simulink model "GNC_physical_diagram"  (R2021b)
settings: Solver=VariableStepAuto  StartTime=0.0  StopTime=10.0  RelTol=1e-3
model workspace (MAT data in the model file):
  AV_Status_Signal = Simulink.Bus
  AV_Status_Signal.Alignment = -1
  AV_Status_Signal.PreserveElementDimensions = 0
  AV_Status_Signal.Elements_internal(1) = Simulink.BusElement
  AV_Status_Signal.Elements_internal(1).DimensionsMode = 'Fixed'
  AV_Status_Signal.Elements_internal(1).SamplingMode = 'Sample based'
  AV_Status_Signal.Elements_internal(1).SampleTime = -1
  AV_Status_Signal.Elements_internal(1).Name = 'Detumbling_Trigger'
  AV_Status_Signal.Elements_internal(1).DataType_internal = 'double'
  AV_Status_Signal.Elements_internal(1).Complexity = 'real'
  AV_Status_Signal.Elements_internal(1).Dimensions = 1
  AV_Status_Signal.Elements_internal(2) = Simulink.BusElement
  AV_Status_Signal.Elements_internal(2).DimensionsMode = 'Fixed'
  AV_Status_Signal.Elements_internal(2).SamplingMode = 'Sample based'
  AV_Status_Signal.Elements_internal(2).SampleTime = -1
  AV_Status_Signal.Elements_internal(2).Name = 'Testing_Trigger'
  AV_Status_Signal.Elements_internal(2).DataType_internal = 'double'
  AV_Status_Signal.Elements_internal(2).Complexity = 'real'
  AV_Status_Signal.Elements_internal(2).Dimensions = 1
  AV_Status_Signal.Elements_internal(3) = Simulink.BusElement
  AV_Status_Signal.Elements_internal(3).DimensionsMode = 'Fixed'
  AV_Status_Signal.Elements_internal(3).SamplingMode = 'Sample based'
  AV_Status_Signal.Elements_internal(3).SampleTime = -1
  AV_Status_Signal.Elements_internal(3).Name = 'Rotation_Trigger'
  AV_Status_Signal.Elements_internal(3).DataType_internal = 'double'
  AV_Status_Signal.Elements_internal(3).Complexity = 'real'
  AV_Status_Signal.Elements_internal(3).Dimensions = 1
  AV_Status_Signal.Elements_internal(4) = Simulink.BusElement
  AV_Status_Signal.Elements_internal(4).DimensionsMode = 'Fixed'
  AV_Status_Signal.Elements_internal(4).SamplingMode = 'Sample based'
  AV_Status_Signal.Elements_internal(4).SampleTime = -1
  AV_Status_Signal.Elements_internal(4).Name = 'Recreation_Trigger'
  AV_Status_Signal.Elements_internal(4).DataType_internal = 'double'
  AV_Status_Signal.Elements_internal(4).Complexity = 'real'
  AV_Status_Signal.Elements_internal(4).Dimensions = 1
  AV_Status_Signal.Elements_internal(5) = Simulink.BusElement
  AV_Status_Signal.Elements_internal(5).DimensionsMode = 'Fixed'
  AV_Status_Signal.Elements_internal(5).SamplingMode = 'Sample based'
  AV_Status_Signal.Elements_internal(5).SampleTime = -1
  AV_Status_Signal.Elements_internal(5).Name = 'Maintain_Trigger'
  AV_Status_Signal.Elements_internal(5).DataType_internal = 'double'
  AV_Status_Signal.Elements_internal(5).Complexity = 'real'
  AV_Status_Signal.Elements_internal(5).Dimensions = 1
  AV_Status_Signal.Elements_internal(6) = Simulink.BusElement
  AV_Status_Signal.Elements_internal(6).DimensionsMode = 'Fixed'
  AV_Status_Signal.Elements_internal(6).SamplingMode = 'Sample based'
  AV_Status_Signal.Elements_internal(6).SampleTime = -1
  AV_Status_Signal.Elements_internal(6).Name = 'End_of_Life_Trigger'
  AV_Status_Signal.Elements_internal(6).DataType_internal = 'double'
  AV_Status_Signal.Elements_internal(6).Complexity = 'real'
  AV_Status_Signal.Elements_internal(6).Dimensions = 1
  AV_Status_Signal.DataScope = 'Auto'
  Actuator_Signal = Simulink.Bus
  Actuator_Signal.Alignment = -1
  Actuator_Signal.PreserveElementDimensions = 0
  Actuator_Signal.Elements_internal(1) = Simulink.BusElement
  Actuator_Signal.Elements_internal(1).DimensionsMode = 'Fixed'
  Actuator_Signal.Elements_internal(1).SamplingMode = 'Sample based'
  Actuator_Signal.Elements_internal(1).SampleTime = -1
  Actuator_Signal.Elements_internal(1).Name = 'Reaction_Wheel_Signal'
  Actuator_Signal.Elements_internal(1).DataType_internal = 'double'
  Actuator_Signal.Elements_internal(1).Complexity = 'real'
  Actuator_Signal.Elements_internal(1).Dimensions = 1
  Actuator_Signal.Elements_internal(2) = Simulink.BusElement
  Actuator_Signal.Elements_internal(2).DimensionsMode = 'Fixed'
  Actuator_Signal.Elements_internal(2).SamplingMode = 'Sample based'
  Actuator_Signal.Elements_internal(2).SampleTime = -1
  Actuator_Signal.Elements_internal(2).Name = 'Magnetorquer_Signal'
  Actuator_Signal.Elements_internal(2).DataType_internal = 'double'
  Actuator_Signal.Elements_internal(2).Complexity = 'real'
  Actuator_Signal.Elements_internal(2).Dimensions = 1
  Actuator_Signal.DataScope = 'Auto'
  Data_Stream = Simulink.Bus
  Data_Stream.Alignment = -1
  Data_Stream.PreserveElementDimensions = 0
  Data_Stream.Elements_internal(1) = Simulink.BusElement
  Data_Stream.Elements_internal(1).DimensionsMode = 'Fixed'
  Data_Stream.Elements_internal(1).SamplingMode = 'Sample based'
  Data_Stream.Elements_internal(1).SampleTime = -1
  Data_Stream.Elements_internal(1).Name = 'State_Estimation_Data'
  Data_Stream.Elements_internal(1).DataType_internal = 'double'
  Data_Stream.Elements_internal(1).Complexity = 'real'
  Data_Stream.Elements_internal(1).Dimensions = 1
  Data_Stream.Elements_internal(2) = Simulink.BusElement
  Data_Stream.Elements_internal(2).DimensionsMode = 'Fixed'
  Data_Stream.Elements_internal(2).SamplingMode = 'Sample based'
  Data_Stream.Elements_internal(2).SampleTime = -1
  Data_Stream.Elements_internal(2).Name = 'Output_Mission_Phases'
  Data_Stream.Elements_internal(2).DataType_internal = 'double'
  Data_Stream.Elements_internal(2).Complexity = 'real'
  Data_Stream.Elements_internal(2).Dimensions = 1
  Data_Stream.Elements_internal(3) = Simulink.BusElement
  Data_Stream.Elements_internal(3).DimensionsMode = 'Fixed'
  Data_Stream.Elements_internal(3).SamplingMode = 'Sample based'
  Data_Stream.Elements_internal(3).SampleTime = -1
  Data_Stream.Elements_internal(3).Name = 'Encoder_Data'
  Data_Stream.Elements_internal(3).DataType_internal = 'double'
  Data_Stream.Elements_internal(3).Complexity = 'real'
  Data_Stream.Elements_internal(3).Dimensions = 1
  Data_Stream.Elements_internal(4) = Simulink.BusElement
  Data_Stream.Elements_internal(4).DimensionsMode = 'Fixed'
  Data_Stream.Elements_internal(4).SamplingMode = 'Sample based'
  Data_Stream.Elements_internal(4).SampleTime = -1
  Data_Stream.Elements_internal(4).Name = 'Sensor_Fusion'
  Data_Stream.Elements_internal(4).DataType_internal = 'double'
  Data_Stream.Elements_internal(4).Complexity = 'real'
  Data_Stream.Elements_internal(4).Dimensions = 1
  Data_Stream.DataScope = 'Auto'
  Magnetororquer_Signal = Simulink.Bus
  Magnetororquer_Signal.Alignment = -1
  Magnetororquer_Signal.PreserveElementDimensions = 0
  Magnetororquer_Signal.Elements_internal(1) = Simulink.BusElement
  Magnetororquer_Signal.Elements_internal(1).DimensionsMode = 'Fixed'
  Magnetororquer_Signal.Elements_internal(1).SamplingMode = 'Sample based'
  Magnetororquer_Signal.Elements_internal(1).SampleTime = -1
  Magnetororquer_Signal.Elements_internal(1).Name = 'Magnetororquer_1_Signal'
  Magnetororquer_Signal.Elements_internal(1).DataType_internal = 'double'
  Magnetororquer_Signal.Elements_internal(1).Complexity = 'real'
  Magnetororquer_Signal.Elements_internal(1).Dimensions = 1
  Magnetororquer_Signal.Elements_internal(2) = Simulink.BusElement
  Magnetororquer_Signal.Elements_internal(2).DimensionsMode = 'Fixed'
  Magnetororquer_Signal.Elements_internal(2).SamplingMode = 'Sample based'
  Magnetororquer_Signal.Elements_internal(2).SampleTime = -1
  Magnetororquer_Signal.Elements_internal(2).Name = 'Magnetororquer_2_Signal'
  Magnetororquer_Signal.Elements_internal(2).DataType_internal = 'double'
  Magnetororquer_Signal.Elements_internal(2).Complexity = 'real'
  Magnetororquer_Signal.Elements_internal(2).Dimensions = 1
  Magnetororquer_Signal.Elements_internal(3) = Simulink.BusElement
  Magnetororquer_Signal.Elements_internal(3).DimensionsMode = 'Fixed'
  Magnetororquer_Signal.Elements_internal(3).SamplingMode = 'Sample based'
  Magnetororquer_Signal.Elements_internal(3).SampleTime = -1
  Magnetororquer_Signal.Elements_internal(3).Name = 'Magnetororquer_3_Signal'
  Magnetororquer_Signal.Elements_internal(3).DataType_internal = 'double'
  Magnetororquer_Signal.Elements_internal(3).Complexity = 'real'
  Magnetororquer_Signal.Elements_internal(3).Dimensions = 1
  Magnetororquer_Signal.Elements_internal(4) = Simulink.BusElement
  Magnetororquer_Signal.Elements_internal(4).DimensionsMode = 'Fixed'
  Magnetororquer_Signal.Elements_internal(4).SamplingMode = 'Sample based'
  Magnetororquer_Signal.Elements_internal(4).SampleTime = -1
  Magnetororquer_Signal.Elements_internal(4).Name = 'Magnetororquer_4_Signal'
  Magnetororquer_Signal.Elements_internal(4).DataType_internal = 'double'
  Magnetororquer_Signal.Elements_internal(4).Complexity = 'real'
  Magnetororquer_Signal.Elements_internal(4).Dimensions = 1
  Magnetororquer_Signal.DataScope = 'Auto'
  Mode_Trigger = Simulink.Bus
  Mode_Trigger.Alignment = -1
  Mode_Trigger.PreserveElementDimensions = 0
  Mode_Trigger.Elements_internal(1) = Simulink.BusElement
  Mode_Trigger.Elements_internal(1).DimensionsMode = 'Fixed'
  Mode_Trigger.Elements_internal(1).SamplingMode = 'Sample based'
  Mode_Trigger.Elements_internal(1).SampleTime = -1
  Mode_Trigger.Elements_internal(1).Name = 'Low_Gravity_Mode_Trigger'
  Mode_Trigger.Elements_internal(1).DataType_internal = 'double'
  Mode_Trigger.Elements_internal(1).Complexity = 'real'
  Mode_Trigger.Elements_internal(1).Dimensions = 1
  Mode_Trigger.Elements_internal(2) = Simulink.BusElement
  Mode_Trigger.Elements_internal(2).DimensionsMode = 'Fixed'
  Mode_Trigger.Elements_internal(2).SamplingMode = 'Sample based'
  Mode_Trigger.Elements_internal(2).SampleTime = -1
  Mode_Trigger.Elements_internal(2).Name = 'High_Gravity_Trigger'
  Mode_Trigger.Elements_internal(2).DataType_internal = 'double'
  Mode_Trigger.Elements_internal(2).Complexity = 'real'
  Mode_Trigger.Elements_internal(2).Dimensions = 1
  Mode_Trigger.Elements_internal(3) = Simulink.BusElement
  Mode_Trigger.Elements_internal(3).DimensionsMode = 'Fixed'
  Mode_Trigger.Elements_internal(3).SamplingMode = 'Sample based'
  Mode_Trigger.Elements_internal(3).SampleTime = -1
  Mode_Trigger.Elements_internal(3).Name = 'Desaturization_Trigger'
  Mode_Trigger.Elements_internal(3).DataType_internal = 'double'
  Mode_Trigger.Elements_internal(3).Complexity = 'real'
  Mode_Trigger.Elements_internal(3).Dimensions = 1
  Mode_Trigger.Elements_internal(4) = Simulink.BusElement
  Mode_Trigger.Elements_internal(4).DimensionsMode = 'Fixed'
  Mode_Trigger.Elements_internal(4).SamplingMode = 'Sample based'
  Mode_Trigger.Elements_internal(4).SampleTime = -1
  Mode_Trigger.Elements_internal(4).Name = 'Safe_Mode_Trigger'
  Mode_Trigger.Elements_internal(4).DataType_internal = 'double'
  Mode_Trigger.Elements_internal(4).Complexity = 'real'
  Mode_Trigger.Elements_internal(4).Dimensions = 1
  Mode_Trigger.Elements_internal(5) = Simulink.BusElement
  Mode_Trigger.Elements_internal(5).DimensionsMode = 'Fixed'
  Mode_Trigger.Elements_internal(5).SamplingMode = 'Sample based'
  Mode_Trigger.Elements_internal(5).SampleTime = -1
  Mode_Trigger.Elements_internal(5).Name = 'Collision_Avoidance_Mode'
  Mode_Trigger.Elements_internal(5).DataType_internal = 'double'
  Mode_Trigger.Elements_internal(5).Complexity = 'real'
  Mode_Trigger.Elements_internal(5).Dimensions = 1
  Mode_Trigger.Elements_internal(6) = Simulink.BusElement
  Mode_Trigger.Elements_internal(6).DimensionsMode = 'Fixed'
  Mode_Trigger.Elements_internal(6).SamplingMode = 'Sample based'
  Mode_Trigger.Elements_internal(6).SampleTime = -1
  Mode_Trigger.Elements_internal(6).Name = 'Idle_Mode_Trigger'
  Mode_Trigger.Elements_internal(6).DataType_internal = 'double'
  Mode_Trigger.Elements_internal(6).Complexity = 'real'
  Mode_Trigger.Elements_internal(6).Dimensions = 1
  Mode_Trigger.DataScope = 'Auto'
  Reaction_Wheel_Signal = Simulink.Bus
  Reaction_Wheel_Signal.Alignment = -1
  Reaction_Wheel_Signal.PreserveElementDimensions = 0
  Reaction_Wheel_Signal.Elements_internal(1) = Simulink.BusElement
  Reaction_Wheel_Signal.Elements_internal(1).DimensionsMode = 'Fixed'
  Reaction_Wheel_Signal.Elements_internal(1).SamplingMode = 'Sample based'
  Reaction_Wheel_Signal.Elements_internal(1).SampleTime = -1
  Reaction_Wheel_Signal.Elements_internal(1).Name = 'Reaction_Wheel_1_Signal'
  Reaction_Wheel_Signal.Elements_internal(1).DataType_internal = 'double'
  Reaction_Wheel_Signal.Elements_internal(1).Complexity = 'real'
  Reaction_Wheel_Signal.Elements_internal(1).Dimensions = 1
  Reaction_Wheel_Signal.Elements_internal(2) = Simulink.BusElement
  Reaction_Wheel_Signal.Elements_internal(2).DimensionsMode = 'Fixed'
  Reaction_Wheel_Signal.Elements_internal(2).SamplingMode = 'Sample based'
  Reaction_Wheel_Signal.Elements_internal(2).SampleTime = -1
  Reaction_Wheel_Signal.Elements_internal(2).Name = 'Reaction_Wheel_2_Signal'
  Reaction_Wheel_Signal.Elements_internal(2).DataType_internal = 'double'
  Reaction_Wheel_Signal.Elements_internal(2).Complexity = 'real'
  Reaction_Wheel_Signal.Elements_internal(2).Dimensions = 1
  Reaction_Wheel_Signal.Elements_internal(3) = Simulink.BusElement
  Reaction_Wheel_Signal.Elements_internal(3).DimensionsMode = 'Fixed'
  Reaction_Wheel_Signal.Elements_internal(3).SamplingMode = 'Sample based'
  Reaction_Wheel_Signal.Elements_internal(3).SampleTime = -1
  Reaction_Wheel_Signal.Elements_internal(3).Name = 'Reaction_Wheel_3_Signal'
  Reaction_Wheel_Signal.Elements_internal(3).DataType_internal = 'double'
  Reaction_Wheel_Signal.Elements_internal(3).Complexity = 'real'
  Reaction_Wheel_Signal.Elements_internal(3).Dimensions = 1
  Reaction_Wheel_Signal.Elements_internal(4) = Simulink.BusElement
  Reaction_Wheel_Signal.Elements_internal(4).DimensionsMode = 'Fixed'
  Reaction_Wheel_Signal.Elements_internal(4).SamplingMode = 'Sample based'
  Reaction_Wheel_Signal.Elements_internal(4).SampleTime = -1
  Reaction_Wheel_Signal.Elements_internal(4).Name = 'Reaction_Wheel_4_Signal'
  Reaction_Wheel_Signal.Elements_internal(4).DataType_internal = 'double'
  Reaction_Wheel_Signal.Elements_internal(4).Complexity = 'real'
  Reaction_Wheel_Signal.Elements_internal(4).Dimensions = 1
  Reaction_Wheel_Signal.DataScope = 'Auto'
  Resources_Budget = Simulink.Bus
  Resources_Budget.Alignment = -1
  Resources_Budget.PreserveElementDimensions = 0
  Resources_Budget.Elements_internal(1) = Simulink.BusElement
  Resources_Budget.Elements_internal(1).DimensionsMode = 'Fixed'
  Resources_Budget.Elements_internal(1).SamplingMode = 'Sample based'
  Resources_Budget.Elements_internal(1).SampleTime = -1
  Resources_Budget.Elements_internal(1).Name = 'Processing_Power'
  Resources_Budget.Elements_internal(1).DataType_internal = 'double'
  Resources_Budget.Elements_internal(1).Complexity = 'real'
  Resources_Budget.Elements_internal(1).Dimensions = 1
  Resources_Budget.Elements_internal(2) = Simulink.BusElement
  Resources_Budget.Elements_internal(2).DimensionsMode = 'Fixed'
  Resources_Budget.Elements_internal(2).SamplingMode = 'Sample based'
  Resources_Budget.Elements_internal(2).SampleTime = -1
  Resources_Budget.Elements_internal(2).Name = 'Memory_Allocation'
  Resources_Budget.Elements_internal(2).DataType_internal = 'double'
  Resources_Budget.Elements_internal(2).Complexity = 'real'
  Resources_Budget.Elements_internal(2).Dimensions = 1
  Resources_Budget.Elements_internal(3) = Simulink.BusElement
  Resources_Budget.Elements_internal(3).DimensionsMode = 'Fixed'
  Resources_Budget.Elements_internal(3).SamplingMode = 'Sample based'
  Resources_Budget.Elements_internal(3).SampleTime = -1
  Resources_Budget.Elements_internal(3).Name = 'Power'
  Resources_Budget.Elements_internal(3).DataType_internal = 'double'
  Resources_Budget.Elements_internal(3).Complexity = 'real'
  Resources_Budget.Elements_internal(3).Dimensions = 1
  Resources_Budget.DataScope = 'Auto'
  Sensor_Health = Simulink.Bus
  Sensor_Health.Alignment = -1
  Sensor_Health.PreserveElementDimensions = 0
  Sensor_Health.Elements_internal(1) = Simulink.BusElement
  Sensor_Health.Elements_internal(1).DimensionsMode = 'Fixed'
  Sensor_Health.Elements_internal(1).SamplingMode = 'Sample based'
  Sensor_Health.Elements_internal(1).SampleTime = -1
  Sensor_Health.Elements_internal(1).Name = 'Sun_Sensor_Health'
  Sensor_Health.Elements_internal(1).DataType_internal = 'double'
  Sensor_Health.Elements_internal(1).Complexity = 'real'
  Sensor_Health.Elements_internal(1).Dimensions = 1
  Sensor_Health.Elements_internal(2) = Simulink.BusElement
  Sensor_Health.Elements_internal(2).DimensionsMode = 'Fixed'
  Sensor_Health.Elements_internal(2).SamplingMode = 'Sample based'
  Sensor_Health.Elements_internal(2).SampleTime = -1
  Sensor_Health.Elements_internal(2).Name = 'IMU_Health'
  Sensor_Health.Elements_internal(2).DataType_internal = 'double'
  Sensor_Health.Elements_internal(2).Complexity = 'real'
  Sensor_Health.Elements_internal(2).Dimensions = 1
  Sensor_Health.Elements_internal(3) = Simulink.BusElement
  Sensor_Health.Elements_internal(3).DimensionsMode = 'Fixed'
  Sensor_Health.Elements_internal(3).SamplingMode = 'Sample based'
  Sensor_Health.Elements_internal(3).SampleTime = -1
  Sensor_Health.Elements_internal(3).Name = 'Magnetometer_Health'
  Sensor_Health.Elements_internal(3).DataType_internal = 'double'
  Sensor_Health.Elements_internal(3).Complexity = 'real'
  Sensor_Health.Elements_internal(3).Dimensions = 1
  Sensor_Health.Elements_internal(4) = Simulink.BusElement
  Sensor_Health.Elements_internal(4).DimensionsMode = 'Fixed'
  Sensor_Health.Elements_internal(4).SamplingMode = 'Sample based'
  Sensor_Health.Elements_internal(4).SampleTime = -1
  Sensor_Health.Elements_internal(4).Name = 'GPS_Health'
  Sensor_Health.Elements_internal(4).DataType_internal = 'double'
  Sensor_Health.Elements_internal(4).Complexity = 'real'
  Sensor_Health.Elements_internal(4).Dimensions = 1
  Sensor_Health.DataScope = 'Auto'
  Sensor_Signal = Simulink.Bus
  Sensor_Signal.Alignment = -1
  Sensor_Signal.PreserveElementDimensions = 0
  Sensor_Signal.Elements_internal(1) = Simulink.BusElement
  Sensor_Signal.Elements_internal(1).DimensionsMode = 'Fixed'
  Sensor_Signal.Elements_internal(1).SamplingMode = 'Sample based'
  Sensor_Signal.Elements_internal(1).SampleTime = -1
  Sensor_Signal.Elements_internal(1).Name = 'Sun_Sensor_Measurment'
  Sensor_Signal.Elements_internal(1).DataType_internal = 'double'
  Sensor_Signal.Elements_internal(1).Complexity = 'real'
  Sensor_Signal.Elements_internal(1).Dimensions = 1
  Sensor_Signal.Elements_internal(2) = Simulink.BusElement
  Sensor_Signal.Elements_internal(2).DimensionsMode = 'Fixed'
  Sensor_Signal.Elements_internal(2).SamplingMode = 'Sample based'
  Sensor_Signal.Elements_internal(2).SampleTime = -1
  Sensor_Signal.Elements_internal(2).Name = 'IMU_Measurement'
  Sensor_Signal.Elements_internal(2).DataType_internal = 'double'
  Sensor_Signal.Elements_internal(2).Complexity = 'real'
  Sensor_Signal.Elements_internal(2).Dimensions = 1
  Sensor_Signal.Elements_internal(3) = Simulink.BusElement
  Sensor_Signal.Elements_internal(3).DimensionsMode = 'Fixed'
  Sensor_Signal.Elements_internal(3).SamplingMode = 'Sample based'
  Sensor_Signal.Elements_internal(3).SampleTime = -1
  Sensor_Signal.Elements_internal(3).Name = 'Magnetometer_Measurement'
  Sensor_Signal.Elements_internal(3).DataType_internal = 'double'
  Sensor_Signal.Elements_internal(3).Complexity = 'real'
  Sensor_Signal.Elements_internal(3).Dimensions = 1
  Sensor_Signal.Elements_internal(4) = Simulink.BusElement
  Sensor_Signal.Elements_internal(4).DimensionsMode = 'Fixed'
  Sensor_Signal.Elements_internal(4).SamplingMode = 'Sample based'
  Sensor_Signal.Elements_internal(4).SampleTime = -1
  Sensor_Signal.Elements_internal(4).Name = 'GPS_Measurement'
  Sensor_Signal.Elements_internal(4).DataType_internal = 'double'
  Sensor_Signal.Elements_internal(4).Complexity = 'real'
  Sensor_Signal.Elements_internal(4).Dimensions = 1
  Sensor_Signal.DataScope = 'Auto'
(part 1 of 2)
settings Model: Creator=jonas  LastModifiedBy=leoba

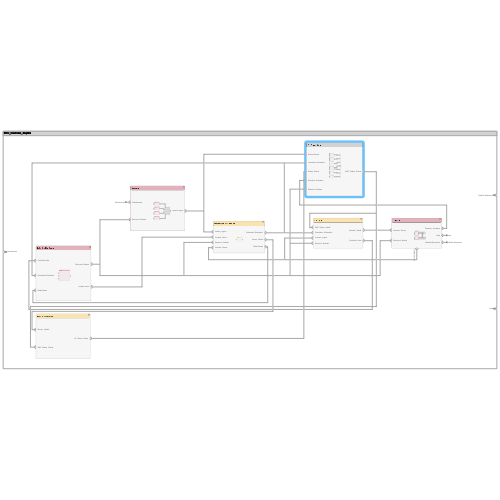
[thumbnail: Simulink's stored preview of the top-level diagram]
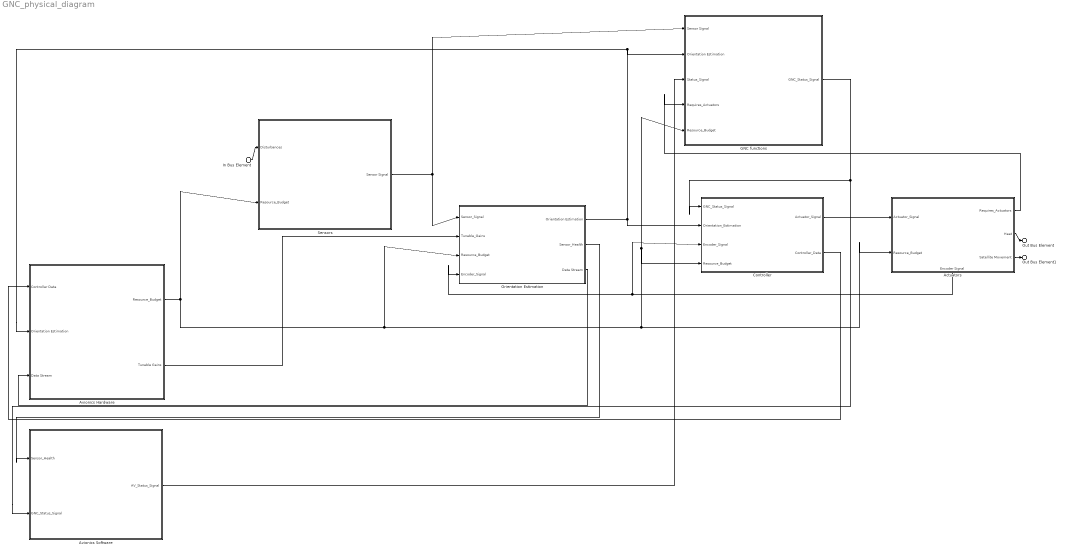
== system GNC_physical_diagram ==
  In Bus Element : Inport  PortName=Disturbances
  Actuators : Subsystem
      settings: PortSchema="{\"entries\":[{\"content\":{\"headerSize\":26,\"margin\":15,\"minimumSpacing\":25,\"sides\":[{\"content\":{\"connectorIds\":[\"In1\",\"In2\"]},\"type\":\"ConnectorPlacement.EquallySpacedRectSide\",\"uuid\":\"4d219d8c-999e-4fa6-ade9-cc6ac14ded32\"},{\"content\":{\"connectorIds\":[\"Out1\",\"Out2\",\"Out3\"],\"side\":\"RIGHT\"},\"type\":\"ConnectorPlacement.EquallySpacedRectSide\",\"uuid\":\"291554bf-cd30-4ae6-93e5-4052e0d4037d\"},{\"content\":{\"connectorIds\":[],\"side\":\"TOP\"},\"type\":\"ConnectorPlacement.EquallySpacedRectSide\",\"uuid\":\"a407b5ba-b8ce-49a8-af7c-64b4689399b6\"},{\"content\":{\"connectorIds\":[\"Out4\"],\"side\":\"BOTTOM\"},\"type\":\"ConnectorPlacement.EquallySpacedRectSide\",\"uuid\":\"28acc806-9e86-4bc6-af71-2b4411156648\"}]},\"type\":\"ConnectorPlacement.EquallySpacedConnector\",\"uuid\":\"1a65b071-c199-4364-8343-b80f4df9252b\"}],\"packageUris\":[\"http://schema.mathworks.com/mf0/Connector/R2020b\"],\"version\":\"1.0\"}"
  Avionics Hardware : Subsystem
      settings: PortSchema="{\"entries\":[{\"content\":{\"headerSize\":26,\"margin\":15,\"minimumSpacing\":25,\"sides\":[{\"content\":{\"connectorIds\":[\"In1\",\"In3\",\"In2\"]},\"type\":\"ConnectorPlacement.EquallySpacedRectSide\",\"uuid\":\"4d219d8c-999e-4fa6-ade9-cc6ac14ded32\"},{\"content\":{\"connectorIds\":[\"Out1\",\"Out2\"],\"side\":\"RIGHT\"},\"type\":\"ConnectorPlacement.EquallySpacedRectSide\",\"uuid\":\"291554bf-cd30-4ae6-93e5-4052e0d4037d\"},{\"content\":{\"connectorIds\":[],\"side\":\"TOP\"},\"type\":\"ConnectorPlacement.EquallySpacedRectSide\",\"uuid\":\"a407b5ba-b8ce-49a8-af7c-64b4689399b6\"},{\"content\":{\"connectorIds\":[],\"side\":\"BOTTOM\"},\"type\":\"ConnectorPlacement.EquallySpacedRectSide\",\"uuid\":\"eed5de48-d554-4a4a-aaed-8ac1beb8b61e\"}]},\"type\":\"ConnectorPlacement.EquallySpacedConnector\",\"uuid\":\"1a65b071-c199-4364-8343-b80f4df9252b\"}],\"packageUris\":[\"http://schema.mathworks.com/mf0/Connector/R2020b\"],\"version\":\"1.0\"}"
  Avionics Software : Subsystem
      settings: PortSchema="{\"entries\":[{\"content\":{\"headerSize\":26,\"margin\":15,\"minimumSpacing\":25,\"sides\":[{\"content\":{\"connectorIds\":[\"In1\",\"In2\"]},\"type\":\"ConnectorPlacement.EquallySpacedRectSide\",\"uuid\":\"9c9f921c-2c3b-482c-ae0a-30fa5cf19172\"},{\"content\":{\"connectorIds\":[\"Out1\"],\"side\":\"RIGHT\"},\"type\":\"ConnectorPlacement.EquallySpacedRectSide\",\"uuid\":\"566c4868-5865-4e1f-981e-d74a35c979c9\"},{\"content\":{\"connectorIds\":[],\"side\":\"TOP\"},\"type\":\"ConnectorPlacement.EquallySpacedRectSide\",\"uuid\":\"2cd88ae2-a2e5-4e25-b817-9d229c73c4c9\"}]},\"type\":\"ConnectorPlacement.EquallySpacedConnector\",\"uuid\":\"48eadbd9-1de4-4fec-af56-45dc4412e923\"}],\"packageUris\":[\"http://schema.mathworks.com/mf0/Connector/R2020b\"],\"version\":\"1.0\"}"
  Controller : Subsystem
      settings: PortSchema="{\"entries\":[{\"content\":{\"headerSize\":26,\"margin\":15,\"minimumSpacing\":25,\"sides\":[{\"content\":{\"connectorIds\":[\"In1\",\"In2\",\"In3\",\"In4\"]},\"type\":\"ConnectorPlacement.EquallySpacedRectSide\",\"uuid\":\"4d219d8c-999e-4fa6-ade9-cc6ac14ded32\"},{\"content\":{\"connectorIds\":[\"Out1\",\"Out2\"],\"side\":\"RIGHT\"},\"type\":\"ConnectorPlacement.EquallySpacedRectSide\",\"uuid\":\"291554bf-cd30-4ae6-93e5-4052e0d4037d\"},{\"content\":{\"connectorIds\":[],\"side\":\"TOP\"},\"type\":\"ConnectorPlacement.EquallySpacedRectSide\",\"uuid\":\"a407b5ba-b8ce-49a8-af7c-64b4689399b6\"}]},\"type\":\"ConnectorPlacement.EquallySpacedConnector\",\"uuid\":\"1a65b071-c199-4364-8343-b80f4df9252b\"}],\"packageUris\":[\"http://schema.mathworks.com/mf0/Connector/R2020b\"],\"version\":\"1.0\"}"
  GNC functions : Subsystem
      settings: PortSchema="{\"entries\":[{\"content\":{\"headerSize\":26,\"margin\":15,\"minimumSpacing\":25,\"sides\":[{\"content\":{\"connectorIds\":[\"In1\",\"In2\",\"In3\",\"In4\",\"In5\"]},\"type\":\"ConnectorPlacement.EquallySpacedRectSide\",\"uuid\":\"9c9f921c-2c3b-482c-ae0a-30fa5cf19172\"},{\"content\":{\"connectorIds\":[\"Out1\"],\"side\":\"RIGHT\"},\"type\":\"ConnectorPlacement.EquallySpacedRectSide\",\"uuid\":\"566c4868-5865-4e1f-981e-d74a35c979c9\"},{\"content\":{\"connectorIds\":[],\"side\":\"TOP\"},\"type\":\"ConnectorPlacement.EquallySpacedRectSide\",\"uuid\":\"2cd88ae2-a2e5-4e25-b817-9d229c73c4c9\"}]},\"type\":\"ConnectorPlacement.EquallySpacedConnector\",\"uuid\":\"48eadbd9-1de4-4fec-af56-45dc4412e923\"}],\"packageUris\":[\"http://schema.mathworks.com/mf0/Connector/R2020b\"],\"version\":\"1.0\"}"
  Orientation Estimation : Subsystem
      settings: PortSchema="{\"entries\":[{\"content\":{\"headerSize\":26,\"margin\":15,\"minimumSpacing\":25,\"sides\":[{\"content\":{\"connectorIds\":[\"In1\",\"In2\",\"In3\",\"In4\"]},\"type\":\"ConnectorPlacement.EquallySpacedRectSide\",\"uuid\":\"4d219d8c-999e-4fa6-ade9-cc6ac14ded32\"},{\"content\":{\"connectorIds\":[\"Out1\",\"Out2\",\"Out3\"],\"side\":\"RIGHT\"},\"type\":\"ConnectorPlacement.EquallySpacedRectSide\",\"uuid\":\"291554bf-cd30-4ae6-93e5-4052e0d4037d\"},{\"content\":{\"connectorIds\":[],\"side\":\"TOP\"},\"type\":\"ConnectorPlacement.EquallySpacedRectSide\",\"uuid\":\"a407b5ba-b8ce-49a8-af7c-64b4689399b6\"}]},\"type\":\"ConnectorPlacement.EquallySpacedConnector\",\"uuid\":\"1a65b071-c199-4364-8343-b80f4df9252b\"}],\"packageUris\":[\"http://schema.mathworks.com/mf0/Connector/R2020b\"],\"version\":\"1.0\"}"
  Sensors : Subsystem
      settings: PortSchema="{\"entries\":[{\"content\":{\"headerSize\":26,\"margin\":15,\"minimumSpacing\":25,\"sides\":[{\"content\":{\"connectorIds\":[\"In1\",\"In2\"]},\"type\":\"ConnectorPlacement.EquallySpacedRectSide\",\"uuid\":\"4d219d8c-999e-4fa6-ade9-cc6ac14ded32\"},{\"content\":{\"connectorIds\":[\"Out1\"],\"side\":\"RIGHT\"},\"type\":\"ConnectorPlacement.EquallySpacedRectSide\",\"uuid\":\"291554bf-cd30-4ae6-93e5-4052e0d4037d\"},{\"content\":{\"connectorIds\":[],\"side\":\"TOP\"},\"type\":\"ConnectorPlacement.EquallySpacedRectSide\",\"uuid\":\"a407b5ba-b8ce-49a8-af7c-64b4689399b6\"}]},\"type\":\"ConnectorPlacement.EquallySpacedConnector\",\"uuid\":\"1a65b071-c199-4364-8343-b80f4df9252b\"}],\"packageUris\":[\"http://schema.mathworks.com/mf0/Connector/R2020b\"],\"version\":\"1.0\"}"
  Out Bus Element1 : Outport  PortName=Satellite Movement
  Out Bus Element : Outport  Port=2  PortName=Heat
  wires:
  Orientation Estimation/1(Orientation Estimation) -> Avionics Hardware/3(Orientation Estimation), GNC functions/2(Orientation Estimation), Controller/2(Orientation_Estimation)
  Orientation Estimation/3(Data Stream) -> Avionics Hardware/2(Data Stream)
  Avionics Hardware/2(Tunable Gains) -> Orientation Estimation/2(Tunable_Gains)
  Controller/1(Actuator_Signal) -> Actuators/1(Actuator_Signal)
  Controller/2(Controller_Data) -> Avionics Hardware/1(Controller Data)
  Actuators/4(Encoder Signal) -> Orientation Estimation/4(Encoder_Signal), Controller/3(Encoder_Signal)
  Actuators/2(Heat) -> Out Bus Element/1
  Actuators/3(Satellite Movement) -> Out Bus Element1/1
  In Bus Element/1 -> Sensors/1(Disturbances)
  Sensors/1(Sensor Signal) -> GNC functions/1(Sensor Signal), Orientation Estimation/1(Sensor_Signal)
  Avionics Software/1(AV_Status_Signal) -> GNC functions/3(Status_Signal)
  Actuators/1(Requires_Actuators) -> GNC functions/4(Requires_Actuators)
  GNC functions/1(GNC_Status_Signal) -> Controller/1(GNC_Status_Signal), Avionics Software/2(GNC_Status_Signal)
  Avionics Hardware/1(Resource_Budget) -> Actuators/2(Resource_Budget), Controller/4(Resource_Budget), GNC functions/5(Resource_Budget), Orientation Estimation/3(Resource_Budget), Sensors/2(Resource_Budget)
  Orientation Estimation/2(Sensor_Health) -> Avionics Software/1(Sensor_Health)

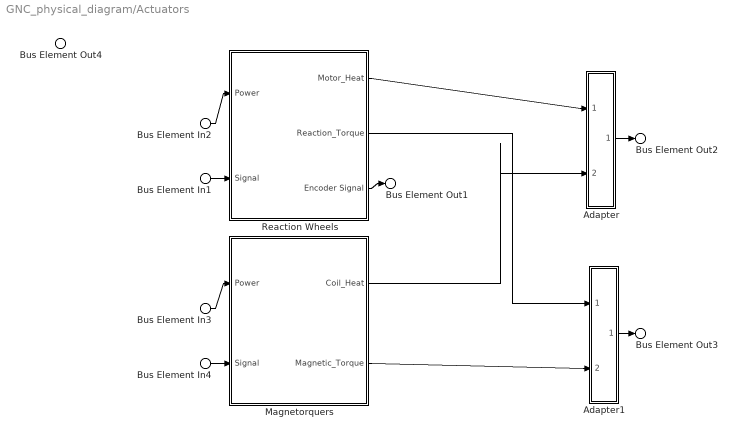
== system GNC_physical_diagram/Actuators ==
  Bus Element In1 : Inport  PortName=Actuator_Signal  Element=Reaction_Wheel_Signal
  Bus Element In4 : Inport  PortName=Actuator_Signal  Element=Magnetorquer_Signal
  Bus Element In2 : Inport  Port=2  PortName=Resource_Budget  Element=Power
  Bus Element In3 : Inport  Port=2  PortName=Resource_Budget  Element=Power
  Adapter : Subsystem
      settings: PortSchema="{\"entries\":[{\"content\":{\"margin\":10,\"minimumSpacing\":15,\"sides\":[{\"content\":{\"connectorIds\":[\"In1\",\"In2\"]},\"type\":\"ConnectorPlacement.EquallySpacedRectSide\",\"uuid\":\"04187947-a540-40f5-bdfb-67f982a6a3c9\"},{\"content\":{\"connectorIds\":[\"Out1\"],\"side\":\"RIGHT\"},\"type\":\"ConnectorPlacement.EquallySpacedRectSide\",\"uuid\":\"f31cf56a-b296-49ce-bb6c-3e31d54897fe\"},{\"content\":{\"connectorIds\":[],\"side\":\"TOP\"},\"type\":\"ConnectorPlacement.EquallySpacedRectSide\",\"uuid\":\"f63c8b68-6d1c-44a5-97b2-14525c5c4754\"}]},\"type\":\"ConnectorPlacement.EquallySpacedConnector\",\"uuid\":\"353cf843-0db6-4928-914d-fdc94187866a\"}],\"packageUris\":[\"http://schema.mathworks.com/mf0/Connector/R2020b\"],\"version\":\"1.0\"}"
  Adapter1 : Subsystem
      settings: PortSchema="{\"entries\":[{\"content\":{\"margin\":10,\"minimumSpacing\":15,\"sides\":[{\"content\":{\"connectorIds\":[\"In1\",\"In2\"]},\"type\":\"ConnectorPlacement.EquallySpacedRectSide\",\"uuid\":\"04187947-a540-40f5-bdfb-67f982a6a3c9\"},{\"content\":{\"connectorIds\":[\"Out1\"],\"side\":\"RIGHT\"},\"type\":\"ConnectorPlacement.EquallySpacedRectSide\",\"uuid\":\"f31cf56a-b296-49ce-bb6c-3e31d54897fe\"},{\"content\":{\"connectorIds\":[],\"side\":\"TOP\"},\"type\":\"ConnectorPlacement.EquallySpacedRectSide\",\"uuid\":\"f63c8b68-6d1c-44a5-97b2-14525c5c4754\"}]},\"type\":\"ConnectorPlacement.EquallySpacedConnector\",\"uuid\":\"353cf843-0db6-4928-914d-fdc94187866a\"}],\"packageUris\":[\"http://schema.mathworks.com/mf0/Connector/R2020b\"],\"version\":\"1.0\"}"
  Magnetorquers : Subsystem
      settings: PortSchema="{\"entries\":[{\"content\":{\"headerSize\":26,\"margin\":15,\"minimumSpacing\":25,\"sides\":[{\"content\":{\"connectorIds\":[\"In1\",\"In2\"]},\"type\":\"ConnectorPlacement.EquallySpacedRectSide\",\"uuid\":\"04187947-a540-40f5-bdfb-67f982a6a3c9\"},{\"content\":{\"connectorIds\":[\"Out1\",\"Out2\"],\"side\":\"RIGHT\"},\"type\":\"ConnectorPlacement.EquallySpacedRectSide\",\"uuid\":\"f31cf56a-b296-49ce-bb6c-3e31d54897fe\"},{\"content\":{\"connectorIds\":[],\"side\":\"TOP\"},\"type\":\"ConnectorPlacement.EquallySpacedRectSide\",\"uuid\":\"f63c8b68-6d1c-44a5-97b2-14525c5c4754\"}]},\"type\":\"ConnectorPlacement.EquallySpacedConnector\",\"uuid\":\"353cf843-0db6-4928-914d-fdc94187866a\"}],\"packageUris\":[\"http://schema.mathworks.com/mf0/Connector/R2020b\"],\"version\":\"1.0\"}"
  Reaction Wheels : Subsystem
      settings: PortSchema="{\"entries\":[{\"content\":{\"headerSize\":26,\"margin\":15,\"minimumSpacing\":25,\"sides\":[{\"content\":{\"connectorIds\":[\"In1\",\"In2\"]},\"type\":\"ConnectorPlacement.EquallySpacedRectSide\",\"uuid\":\"04187947-a540-40f5-bdfb-67f982a6a3c9\"},{\"content\":{\"connectorIds\":[\"Out1\",\"Out2\",\"Out3\"],\"side\":\"RIGHT\"},\"type\":\"ConnectorPlacement.EquallySpacedRectSide\",\"uuid\":\"f31cf56a-b296-49ce-bb6c-3e31d54897fe\"},{\"content\":{\"connectorIds\":[],\"side\":\"TOP\"},\"type\":\"ConnectorPlacement.EquallySpacedRectSide\",\"uuid\":\"f63c8b68-6d1c-44a5-97b2-14525c5c4754\"}]},\"type\":\"ConnectorPlacement.EquallySpacedConnector\",\"uuid\":\"353cf843-0db6-4928-914d-fdc94187866a\"}],\"packageUris\":[\"http://schema.mathworks.com/mf0/Connector/R2020b\"],\"version\":\"1.0\"}"
  Bus Element Out4 : Outport  PortName=Requires_Actuators
  Bus Element Out2 : Outport  Port=2  PortName=Heat
  Bus Element Out3 : Outport  Port=3  PortName=Satellite Movement
  Bus Element Out1 : Outport  Port=4  PortName=Encoder Signal
  wires:
  Adapter/1(Heat) -> Bus Element Out2/1
  Reaction Wheels/1(Motor_Heat) -> Adapter/1(Motor_Heat)
  Magnetorquers/1(Coil_Heat) -> Adapter/2(Coil_Heat)
  Bus Element In2/1 -> Reaction Wheels/1(Power)
  Bus Element In3/1 -> Magnetorquers/1(Power)
  Adapter1/1(Satellite Movement) -> Bus Element Out3/1
  Reaction Wheels/2(Reaction_Torque) -> Adapter1/1(Reaction_Torque)
  Magnetorquers/2(Magnetic_Torque) -> Adapter1/2(Magnetic_Torque)
  Reaction Wheels/3(Encoder Signal) -> Bus Element Out1/1
  Bus Element In1/1 -> Reaction Wheels/2(Signal)
  Bus Element In4/1 -> Magnetorquers/2(Signal)

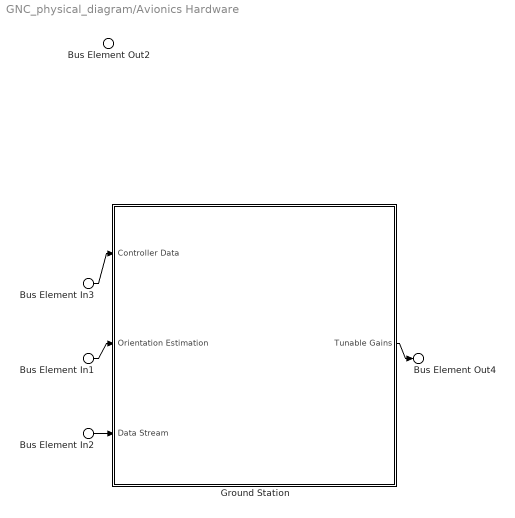
== system GNC_physical_diagram/Avionics Hardware ==
  Bus Element In3 : Inport  PortName=Controller Data
  Bus Element In2 : Inport  Port=2  PortName=Data Stream
  Bus Element In1 : Inport  Port=3  PortName=Orientation Estimation
  Ground Station : Subsystem
      settings: PortSchema="{\"entries\":[{\"content\":{\"headerSize\":26,\"margin\":15,\"minimumSpacing\":25,\"sides\":[{\"content\":{\"connectorIds\":[\"In1\",\"In2\",\"In3\"]},\"type\":\"ConnectorPlacement.EquallySpacedRectSide\",\"uuid\":\"3fbe4e58-7602-4c86-a4ec-d961853d330a\"},{\"content\":{\"connectorIds\":[\"Out1\"],\"side\":\"RIGHT\"},\"type\":\"ConnectorPlacement.EquallySpacedRectSide\",\"uuid\":\"06672cb8-3b8e-4839-b0cd-02d4db3e65cc\"},{\"content\":{\"connectorIds\":[],\"side\":\"TOP\"},\"type\":\"ConnectorPlacement.EquallySpacedRectSide\",\"uuid\":\"be669827-c1af-47c0-a821-253fc1527860\"}]},\"type\":\"ConnectorPlacement.EquallySpacedConnector\",\"uuid\":\"0440c43f-f42b-4dc1-9ac4-21f010a67c28\"}],\"packageUris\":[\"http://schema.mathworks.com/mf0/Connector/R2020b\"],\"version\":\"1.0\"}"
  Bus Element Out2 : Outport  PortName=Resource_Budget
  Bus Element Out4 : Outport  Port=2  PortName=Tunable Gains
  wires:
  Ground Station/1(Tunable Gains) -> Bus Element Out4/1
  Bus Element In3/1 -> Ground Station/1(Controller Data)
  Bus Element In1/1 -> Ground Station/2(Orientation Estimation)
  Bus Element In2/1 -> Ground Station/3(Data Stream)

== system GNC_physical_diagram/Avionics Software ==
  Bus Element In2 : Inport  PortName=Sensor_Health
  Bus Element In1 : Inport  Port=2  PortName=GNC_Status_Signal
  Bus Element Out1 : Outport  PortName=AV_Status_Signal

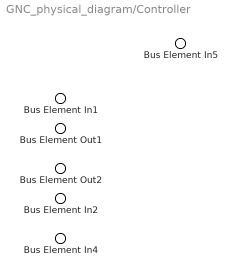
== system GNC_physical_diagram/Controller ==
  Bus Element In5 : Inport  PortName=GNC_Status_Signal
  Bus Element In1 : Inport  Port=2  PortName=Orientation_Estimation
  Bus Element In2 : Inport  Port=3  PortName=Encoder_Signal
  Bus Element In4 : Inport  Port=4  PortName=Resource_Budget
  Bus Element Out1 : Outport  PortName=Actuator_Signal
  Bus Element Out2 : Outport  Port=2  PortName=Controller_Data

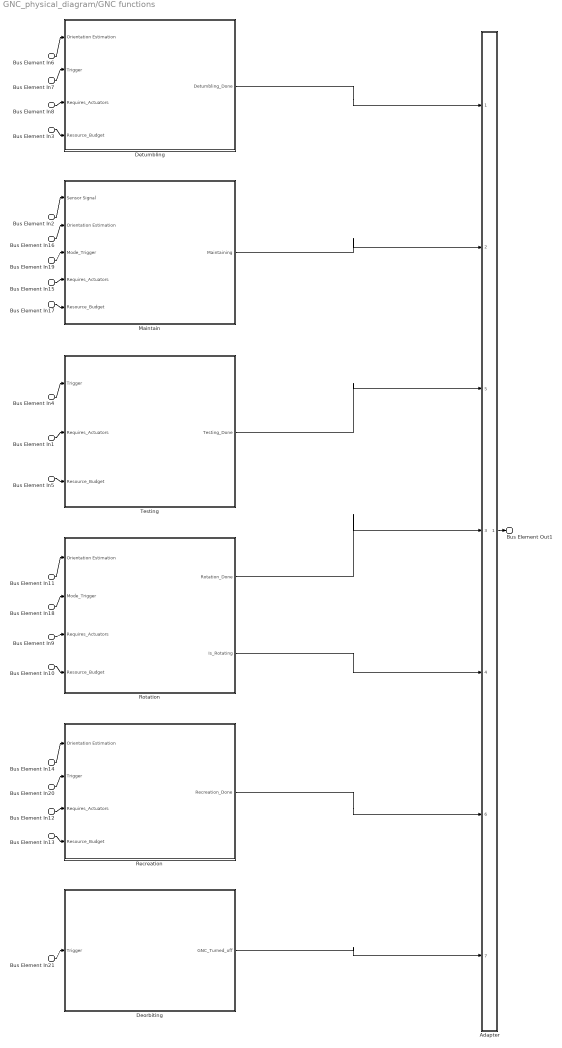
== system GNC_physical_diagram/GNC functions ==
  Bus Element In2 : Inport  PortName=Sensor Signal
  Bus Element In{6,11,14,16} (4 alike) : Inport  Port=2  PortName=Orientation Estimation
  Bus Element In7 : Inport  Port=3  PortName=Status_Signal  Element=Detumbling_Trigger
  Bus Element In4 : Inport  Port=3  PortName=Status_Signal  Element=Testing_Trigger
  Bus Element In18 : Inport  Port=3  PortName=Status_Signal  Element=Rotation_Trigger
  Bus Element In20 : Inport  Port=3  PortName=Status_Signal  Element=Recreation_Trigger
  Bus Element In19 : Inport  Port=3  PortName=Status_Signal  Element=Maintain_Trigger
  Bus Element In21 : Inport  Port=3  PortName=Status_Signal  Element=End_of_Life_Trigger
  Bus Element In{1,8..9,12,15} (5 alike) : Inport  Port=4  PortName=Requires_Actuators
  Bus Element In{3,5,10,13,17} (5 alike) : Inport  Port=5  PortName=Resource_Budget
  Adapter : Subsystem
      settings: PortSchema="{\"entries\":[{\"content\":{\"margin\":10,\"minimumSpacing\":15,\"sides\":[{\"content\":{\"connectorIds\":[\"In1\",\"In2\",\"In5\",\"In3\",\"In4\",\"In6\",\"In7\"]},\"type\":\"ConnectorPlacement.EquallySpacedRectSide\",\"uuid\":\"9c9f921c-2c3b-482c-ae0a-30fa5cf19172\"},{\"content\":{\"connectorIds\":[\"Out1\"],\"side\":\"RIGHT\"},\"type\":\"ConnectorPlacement.EquallySpacedRectSide\",\"uuid\":\"566c4868-5865-4e1f-981e-d74a35c979c9\"},{\"content\":{\"connectorIds\":[],\"side\":\"TOP\"},\"type\":\"ConnectorPlacement.EquallySpacedRectSide\",\"uuid\":\"2cd88ae2-a2e5-4e25-b817-9d229c73c4c9\"}]},\"type\":\"ConnectorPlacement.EquallySpacedConnector\",\"uuid\":\"48eadbd9-1de4-4fec-af56-45dc4412e923\"}],\"packageUris\":[\"http://schema.mathworks.com/mf0/Connector/R2020b\"],\"version\":\"1.0\"}"
  Deorbiting : Subsystem
      settings: PortSchema="{\"entries\":[{\"content\":{\"headerSize\":26,\"margin\":15,\"minimumSpacing\":25,\"sides\":[{\"content\":{\"connectorIds\":[\"In1\"]},\"type\":\"ConnectorPlacement.EquallySpacedRectSide\",\"uuid\":\"9c9f921c-2c3b-482c-ae0a-30fa5cf19172\"},{\"content\":{\"connectorIds\":[\"Out1\"],\"side\":\"RIGHT\"},\"type\":\"ConnectorPlacement.EquallySpacedRectSide\",\"uuid\":\"566c4868-5865-4e1f-981e-d74a35c979c9\"},{\"content\":{\"connectorIds\":[],\"side\":\"TOP\"},\"type\":\"ConnectorPlacement.EquallySpacedRectSide\",\"uuid\":\"2cd88ae2-a2e5-4e25-b817-9d229c73c4c9\"}]},\"type\":\"ConnectorPlacement.EquallySpacedConnector\",\"uuid\":\"48eadbd9-1de4-4fec-af56-45dc4412e923\"}],\"packageUris\":[\"http://schema.mathworks.com/mf0/Connector/R2020b\"],\"version\":\"1.0\"}"
  Detumbling : Subsystem
      settings: PortSchema="{\"entries\":[{\"content\":{\"headerSize\":26,\"margin\":15,\"minimumSpacing\":25,\"sides\":[{\"content\":{\"connectorIds\":[\"In1\",\"In2\",\"In3\",\"In4\"]},\"type\":\"ConnectorPlacement.EquallySpacedRectSide\",\"uuid\":\"9c9f921c-2c3b-482c-ae0a-30fa5cf19172\"},{\"content\":{\"connectorIds\":[\"Out1\"],\"side\":\"RIGHT\"},\"type\":\"ConnectorPlacement.EquallySpacedRectSide\",\"uuid\":\"566c4868-5865-4e1f-981e-d74a35c979c9\"},{\"content\":{\"connectorIds\":[],\"side\":\"TOP\"},\"type\":\"ConnectorPlacement.EquallySpacedRectSide\",\"uuid\":\"2cd88ae2-a2e5-4e25-b817-9d229c73c4c9\"}]},\"type\":\"ConnectorPlacement.EquallySpacedConnector\",\"uuid\":\"48eadbd9-1de4-4fec-af56-45dc4412e923\"}],\"packageUris\":[\"http://schema.mathworks.com/mf0/Connector/R2020b\"],\"version\":\"1.0\"}"
  Maintain : Subsystem
      settings: PortSchema="{\"entries\":[{\"content\":{\"headerSize\":26,\"margin\":15,\"minimumSpacing\":25,\"sides\":[{\"content\":{\"connectorIds\":[\"In1\",\"In2\",\"In3\",\"In4\",\"In5\"]},\"type\":\"ConnectorPlacement.EquallySpacedRectSide\",\"uuid\":\"9c9f921c-2c3b-482c-ae0a-30fa5cf19172\"},{\"content\":{\"connectorIds\":[\"Out1\"],\"side\":\"RIGHT\"},\"type\":\"ConnectorPlacement.EquallySpacedRectSide\",\"uuid\":\"566c4868-5865-4e1f-981e-d74a35c979c9\"},{\"content\":{\"connectorIds\":[],\"side\":\"TOP\"},\"type\":\"ConnectorPlacement.EquallySpacedRectSide\",\"uuid\":\"2cd88ae2-a2e5-4e25-b817-9d229c73c4c9\"}]},\"type\":\"ConnectorPlacement.EquallySpacedConnector\",\"uuid\":\"48eadbd9-1de4-4fec-af56-45dc4412e923\"}],\"packageUris\":[\"http://schema.mathworks.com/mf0/Connector/R2020b\"],\"version\":\"1.0\"}"
  Recreation : Subsystem
      settings: PortSchema="{\"entries\":[{\"content\":{\"headerSize\":26,\"margin\":15,\"minimumSpacing\":25,\"sides\":[{\"content\":{\"connectorIds\":[\"In1\",\"In2\",\"In3\",\"In4\"]},\"type\":\"ConnectorPlacement.EquallySpacedRectSide\",\"uuid\":\"9c9f921c-2c3b-482c-ae0a-30fa5cf19172\"},{\"content\":{\"connectorIds\":[\"Out1\"],\"side\":\"RIGHT\"},\"type\":\"ConnectorPlacement.EquallySpacedRectSide\",\"uuid\":\"566c4868-5865-4e1f-981e-d74a35c979c9\"},{\"content\":{\"connectorIds\":[],\"side\":\"TOP\"},\"type\":\"ConnectorPlacement.EquallySpacedRectSide\",\"uuid\":\"2cd88ae2-a2e5-4e25-b817-9d229c73c4c9\"}]},\"type\":\"ConnectorPlacement.EquallySpacedConnector\",\"uuid\":\"48eadbd9-1de4-4fec-af56-45dc4412e923\"}],\"packageUris\":[\"http://schema.mathworks.com/mf0/Connector/R2020b\"],\"version\":\"1.0\"}"
  Rotation : Subsystem
      settings: PortSchema="{\"entries\":[{\"content\":{\"headerSize\":26,\"margin\":15,\"minimumSpacing\":25,\"sides\":[{\"content\":{\"connectorIds\":[\"In1\",\"In2\",\"In3\",\"In4\"]},\"type\":\"ConnectorPlacement.EquallySpacedRectSide\",\"uuid\":\"9c9f921c-2c3b-482c-ae0a-30fa5cf19172\"},{\"content\":{\"connectorIds\":[\"Out1\",\"Out2\"],\"side\":\"RIGHT\"},\"type\":\"ConnectorPlacement.EquallySpacedRectSide\",\"uuid\":\"566c4868-5865-4e1f-981e-d74a35c979c9\"},{\"content\":{\"connectorIds\":[],\"side\":\"TOP\"},\"type\":\"ConnectorPlacement.EquallySpacedRectSide\",\"uuid\":\"2cd88ae2-a2e5-4e25-b817-9d229c73c4c9\"}]},\"type\":\"ConnectorPlacement.EquallySpacedConnector\",\"uuid\":\"48eadbd9-1de4-4fec-af56-45dc4412e923\"}],\"packageUris\":[\"http://schema.mathworks.com/mf0/Connector/R2020b\"],\"version\":\"1.0\"}"
  Testing : Subsystem
      settings: PortSchema="{\"entries\":[{\"content\":{\"headerSize\":26,\"margin\":15,\"minimumSpacing\":25,\"sides\":[{\"content\":{\"connectorIds\":[\"In1\",\"In2\",\"In3\"]},\"type\":\"ConnectorPlacement.EquallySpacedRectSide\",\"uuid\":\"9c9f921c-2c3b-482c-ae0a-30fa5cf19172\"},{\"content\":{\"connectorIds\":[\"Out1\"],\"side\":\"RIGHT\"},\"type\":\"ConnectorPlacement.EquallySpacedRectSide\",\"uuid\":\"566c4868-5865-4e1f-981e-d74a35c979c9\"},{\"content\":{\"connectorIds\":[],\"side\":\"TOP\"},\"type\":\"ConnectorPlacement.EquallySpacedRectSide\",\"uuid\":\"2cd88ae2-a2e5-4e25-b817-9d229c73c4c9\"}]},\"type\":\"ConnectorPlacement.EquallySpacedConnector\",\"uuid\":\"48eadbd9-1de4-4fec-af56-45dc4412e923\"}],\"packageUris\":[\"http://schema.mathworks.com/mf0/Connector/R2020b\"],\"version\":\"1.0\"}"
  Bus Element Out1 : Outport  PortName=GNC_Status_Signal
  wires:
  Bus Element In6/1 -> Detumbling/1(Orientation Estimation)
  Bus Element In7/1 -> Detumbling/2(Trigger)
  Bus Element In8/1 -> Detumbling/3(Requires_Actuators)
  Detumbling/1(Detumbling_Done) -> Adapter/1(Detumbling_Done)
  Rotation/1(Rotation_Done) -> Adapter/3(Rotation_Done)
  Rotation/2(Is_Rotating) -> Adapter/4(Is_Rotating)
  Adapter/1(GNC_Status_) -> Bus Element Out1/1
  Bus Element In3/1 -> Detumbling/4(Resource_Budget)
  Testing/1(Testing_Done) -> Adapter/5(Testing_Done)
  Bus Element In4/1 -> Testing/1(Trigger)
  Bus Element In5/1 -> Testing/3(Resource_Budget)
  Bus Element In9/1 -> Rotation/3(Requires_Actuators)
  Bus Element In10/1 -> Rotation/4(Resource_Budget)
  Bus Element In11/1 -> Rotation/1(Orientation Estimation)
  Bus Element In12/1 -> Recreation/3(Requires_Actuators)
  Bus Element In13/1 -> Recreation/4(Resource_Budget)
  Bus Element In14/1 -> Recreation/1(Orientation Estimation)
  Bus Element In15/1 -> Maintain/4(Requires_Actuators)
  Bus Element In16/1 -> Maintain/2(Orientation Estimation)
  Bus Element In2/1 -> Maintain/1(Sensor Signal)
  Maintain/1(Maintaining) -> Adapter/2(Maintaining)
  Bus Element In17/1 -> Maintain/5(Resource_Budget)
  Bus Element In18/1 -> Rotation/2(Mode_Trigger)
  Bus Element In20/1 -> Recreation/2(Trigger)
  Recreation/1(Recreation_Done) -> Adapter/6(Recreation_Done)
  Bus Element In19/1 -> Maintain/3(Mode_Trigger)
  Bus Element In21/1 -> Deorbiting/1(Trigger)
  Deorbiting/1(GNC_Turned_off) -> Adapter/7(GNC_Turned_off)
  Bus Element In1/1 -> Testing/2(Requires_Actuators)

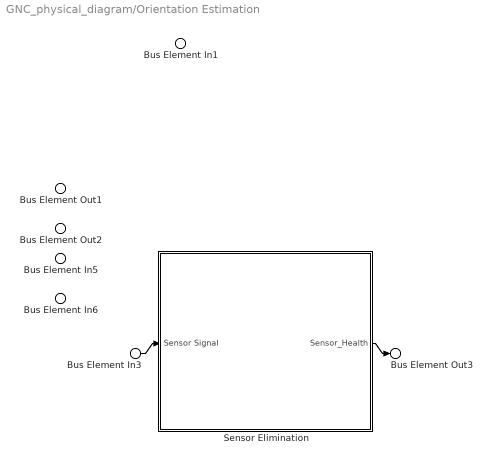
== system GNC_physical_diagram/Orientation Estimation ==
  Bus Element In3 : Inport  PortName=Sensor_Signal
  Bus Element In5 : Inport  Port=2  PortName=Tunable_Gains
  Bus Element In1 : Inport  Port=3  PortName=Resource_Budget
  Bus Element In6 : Inport  Port=4  PortName=Encoder_Signal
  Sensor Elimination : Subsystem
      settings: PortSchema="{\"entries\":[{\"content\":{\"headerSize\":26,\"margin\":15,\"minimumSpacing\":25,\"sides\":[{\"content\":{\"connectorIds\":[\"In1\"]},\"type\":\"ConnectorPlacement.EquallySpacedRectSide\",\"uuid\":\"84b5d53f-2022-465e-8fea-a5f6f770027c\"},{\"content\":{\"connectorIds\":[\"Out1\"],\"side\":\"RIGHT\"},\"type\":\"ConnectorPlacement.EquallySpacedRectSide\",\"uuid\":\"3040b22b-4da9-4e90-8b1d-cb2b07104062\"},{\"content\":{\"connectorIds\":[],\"side\":\"TOP\"},\"type\":\"ConnectorPlacement.EquallySpacedRectSide\",\"uuid\":\"0c703596-6fc3-4e59-bd9e-7a374b07bd61\"}]},\"type\":\"ConnectorPlacement.EquallySpacedConnector\",\"uuid\":\"5254ac91-cce0-48ff-acfe-a25b2e5a66da\"}],\"packageUris\":[\"http://schema.mathworks.com/mf0/Connector/R2020b\"],\"version\":\"1.0\"}"
  Bus Element Out1 : Outport  PortName=Orientation Estimation
  Bus Element Out3 : Outport  Port=2  PortName=Sensor_Health
  Bus Element Out2 : Outport  Port=3  PortName=Data Stream
  wires:
  Bus Element In3/1 -> Sensor Elimination/1(Sensor Signal)
  Sensor Elimination/1(Sensor_Health) -> Bus Element Out3/1

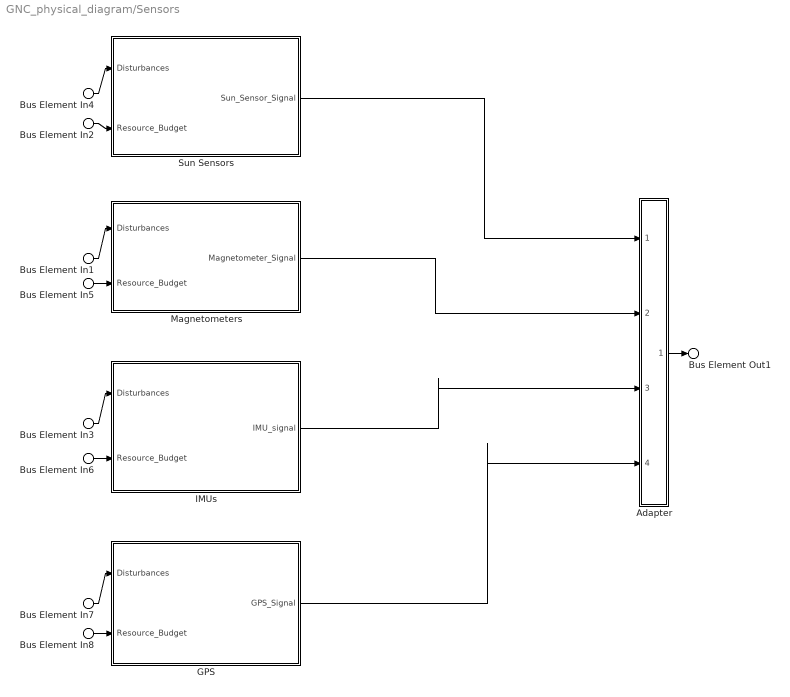
== system GNC_physical_diagram/Sensors ==
  Bus Element In{1,3..4,7} (4 alike) : Inport  PortName=Disturbances
  Bus Element In{2,5..6,8} (4 alike) : Inport  Port=2  PortName=Resource_Budget
  Adapter : Subsystem
      settings: PortSchema="{\"entries\":[{\"content\":{\"margin\":10,\"minimumSpacing\":15,\"sides\":[{\"content\":{\"connectorIds\":[\"In1\",\"In2\",\"In3\",\"In4\"]},\"type\":\"ConnectorPlacement.EquallySpacedRectSide\",\"uuid\":\"0d9fb8ed-dc34-468d-b76e-34d51d64a929\"},{\"content\":{\"connectorIds\":[\"Out1\"],\"side\":\"RIGHT\"},\"type\":\"ConnectorPlacement.EquallySpacedRectSide\",\"uuid\":\"3640ebdc-29ef-4736-b1f3-b11a5268a051\"},{\"content\":{\"connectorIds\":[],\"side\":\"TOP\"},\"type\":\"ConnectorPlacement.EquallySpacedRectSide\",\"uuid\":\"ee7dc95f-9ee4-4519-b423-ed00e53cf3e5\"}]},\"type\":\"ConnectorPlacement.EquallySpacedConnector\",\"uuid\":\"5502122b-b863-467a-b80b-8b9d26248ea6\"}],\"packageUris\":[\"http://schema.mathworks.com/mf0/Connector/R2020b\"],\"version\":\"1.0\"}"
  GPS : Subsystem
      settings: PortSchema="{\"entries\":[{\"content\":{\"headerSize\":26,\"margin\":15,\"minimumSpacing\":25,\"sides\":[{\"content\":{\"connectorIds\":[\"In1\",\"In2\"]},\"type\":\"ConnectorPlacement.EquallySpacedRectSide\",\"uuid\":\"84b5d53f-2022-465e-8fea-a5f6f770027c\"},{\"content\":{\"connectorIds\":[\"Out1\"],\"side\":\"RIGHT\"},\"type\":\"ConnectorPlacement.EquallySpacedRectSide\",\"uuid\":\"3040b22b-4da9-4e90-8b1d-cb2b07104062\"},{\"content\":{\"connectorIds\":[],\"side\":\"TOP\"},\"type\":\"ConnectorPlacement.EquallySpacedRectSide\",\"uuid\":\"0c703596-6fc3-4e59-bd9e-7a374b07bd61\"}]},\"type\":\"ConnectorPlacement.EquallySpacedConnector\",\"uuid\":\"5254ac91-cce0-48ff-acfe-a25b2e5a66da\"}],\"packageUris\":[\"http://schema.mathworks.com/mf0/Connector/R2020b\"],\"version\":\"1.0\"}"
  IMUs : Subsystem
      settings: PortSchema="{\"entries\":[{\"content\":{\"headerSize\":26,\"margin\":15,\"minimumSpacing\":25,\"sides\":[{\"content\":{\"connectorIds\":[\"In1\",\"In2\"]},\"type\":\"ConnectorPlacement.EquallySpacedRectSide\",\"uuid\":\"0d9fb8ed-dc34-468d-b76e-34d51d64a929\"},{\"content\":{\"connectorIds\":[\"Out1\"],\"side\":\"RIGHT\"},\"type\":\"ConnectorPlacement.EquallySpacedRectSide\",\"uuid\":\"3640ebdc-29ef-4736-b1f3-b11a5268a051\"},{\"content\":{\"connectorIds\":[],\"side\":\"TOP\"},\"type\":\"ConnectorPlacement.EquallySpacedRectSide\",\"uuid\":\"ee7dc95f-9ee4-4519-b423-ed00e53cf3e5\"}]},\"type\":\"ConnectorPlacement.EquallySpacedConnector\",\"uuid\":\"5502122b-b863-467a-b80b-8b9d26248ea6\"}],\"packageUris\":[\"http://schema.mathworks.com/mf0/Connector/R2020b\"],\"version\":\"1.0\"}"
  Magnetometers : Subsystem
      settings: PortSchema="{\"entries\":[{\"content\":{\"headerSize\":26,\"margin\":15,\"minimumSpacing\":25,\"sides\":[{\"content\":{\"connectorIds\":[\"In1\",\"In2\"]},\"type\":\"ConnectorPlacement.EquallySpacedRectSide\",\"uuid\":\"0d9fb8ed-dc34-468d-b76e-34d51d64a929\"},{\"content\":{\"connectorIds\":[\"Out1\"],\"side\":\"RIGHT\"},\"type\":\"ConnectorPlacement.EquallySpacedRectSide\",\"uuid\":\"3640ebdc-29ef-4736-b1f3-b11a5268a051\"},{\"content\":{\"connectorIds\":[],\"side\":\"TOP\"},\"type\":\"ConnectorPlacement.EquallySpacedRectSide\",\"uuid\":\"ee7dc95f-9ee4-4519-b423-ed00e53cf3e5\"}]},\"type\":\"ConnectorPlacement.EquallySpacedConnector\",\"uuid\":\"5502122b-b863-467a-b80b-8b9d26248ea6\"}],\"packageUris\":[\"http://schema.mathworks.com/mf0/Connector/R2020b\"],\"version\":\"1.0\"}"
  Sun Sensors : Subsystem
      settings: PortSchema="{\"entries\":[{\"content\":{\"headerSize\":26,\"margin\":15,\"minimumSpacing\":25,\"sides\":[{\"content\":{\"connectorIds\":[\"In1\",\"In2\"]},\"type\":\"ConnectorPlacement.EquallySpacedRectSide\",\"uuid\":\"0d9fb8ed-dc34-468d-b76e-34d51d64a929\"},{\"content\":{\"connectorIds\":[\"Out1\"],\"side\":\"RIGHT\"},\"type\":\"ConnectorPlacement.EquallySpacedRectSide\",\"uuid\":\"3640ebdc-29ef-4736-b1f3-b11a5268a051\"},{\"content\":{\"connectorIds\":[],\"side\":\"TOP\"},\"type\":\"ConnectorPlacement.EquallySpacedRectSide\",\"uuid\":\"ee7dc95f-9ee4-4519-b423-ed00e53cf3e5\"}]},\"type\":\"ConnectorPlacement.EquallySpacedConnector\",\"uuid\":\"5502122b-b863-467a-b80b-8b9d26248ea6\"}],\"packageUris\":[\"http://schema.mathworks.com/mf0/Connector/R2020b\"],\"version\":\"1.0\"}"
  Bus Element Out1 : Outport  PortName=Sensor Signal
  wires:
  Sun Sensors/1(Sun_Sensor_Signal) -> Adapter/1(Sun_Sensor_Signal)
  Adapter/1(Sensor Signal) -> Bus Element Out1/1
  Magnetometers/1(Magnetometer_Signal) -> Adapter/2(Magnetometer_Signal)
  IMUs/1(IMU_signal) -> Adapter/3(IMU_signal)
  Bus Element In4/1 -> Sun Sensors/1(Disturbances)
  Bus Element In1/1 -> Magnetometers/1(Disturbances)
  Bus Element In3/1 -> IMUs/1(Disturbances)
  Bus Element In2/1 -> Sun Sensors/2(Resource_Budget)
  Bus Element In5/1 -> Magnetometers/2(Resource_Budget)
  Bus Element In6/1 -> IMUs/2(Resource_Budget)
  GPS/1(GPS_Signal) -> Adapter/4(GPS_Signal)
  Bus Element In7/1 -> GPS/1(Disturbances)
  Bus Element In8/1 -> GPS/2(Resource_Budget)

== system GNC_physical_diagram/Actuators/Adapter ==
  In Bus Element : Inport  PortName=Motor_Heat
  Bus Element In2 : Inport  Port=2  PortName=Coil_Heat
  Out Bus Element : Outport  PortName=Heat
  wires:
  In Bus Element/1 -> Out Bus Element/1

== system GNC_physical_diagram/Actuators/Adapter1 ==
  In Bus Element : Inport  PortName=Reaction_Torque
  Bus Element In2 : Inport  Port=2  PortName=Magnetic_Torque
  Out Bus Element : Outport  PortName=Satellite Movement
  wires:
  In Bus Element/1 -> Out Bus Element/1

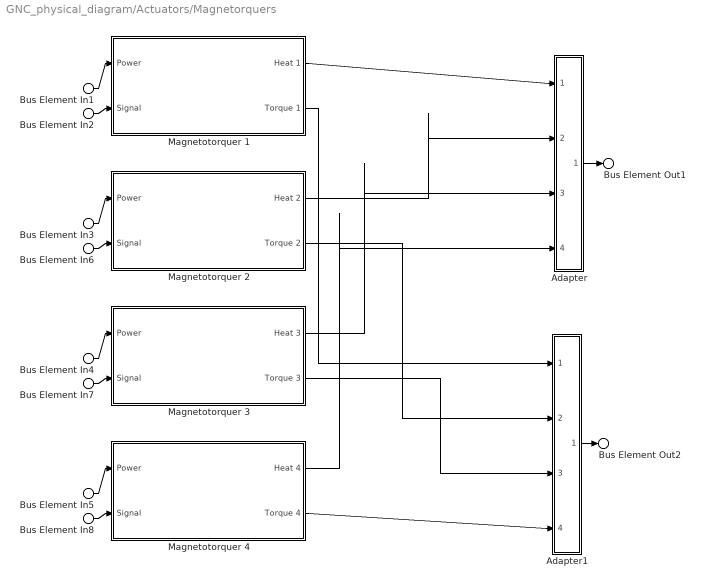
== system GNC_physical_diagram/Actuators/Magnetorquers ==
  Bus Element In{1,3..5} (4 alike) : Inport  PortName=Power
  Bus Element In2 : Inport  Port=2  PortName=Signal  Element=Magnetororquer_1_Signal
  Bus Element In6 : Inport  Port=2  PortName=Signal  Element=Magnetororquer_2_Signal
  Bus Element In7 : Inport  Port=2  PortName=Signal  Element=Magnetororquer_3_Signal
  Bus Element In8 : Inport  Port=2  PortName=Signal  Element=Magnetororquer_4_Signal
  Adapter : Subsystem
      settings: PortSchema="{\"entries\":[{\"content\":{\"margin\":10,\"minimumSpacing\":15,\"sides\":[{\"content\":{\"connectorIds\":[\"In1\",\"In2\",\"In3\",\"In4\"]},\"type\":\"ConnectorPlacement.EquallySpacedRectSide\",\"uuid\":\"0d9fb8ed-dc34-468d-b76e-34d51d64a929\"},{\"content\":{\"connectorIds\":[\"Out1\"],\"side\":\"RIGHT\"},\"type\":\"ConnectorPlacement.EquallySpacedRectSide\",\"uuid\":\"3640ebdc-29ef-4736-b1f3-b11a5268a051\"},{\"content\":{\"connectorIds\":[],\"side\":\"TOP\"},\"type\":\"ConnectorPlacement.EquallySpacedRectSide\",\"uuid\":\"ee7dc95f-9ee4-4519-b423-ed00e53cf3e5\"}]},\"type\":\"ConnectorPlacement.EquallySpacedConnector\",\"uuid\":\"5502122b-b863-467a-b80b-8b9d26248ea6\"}],\"packageUris\":[\"http://schema.mathworks.com/mf0/Connector/R2020b\"],\"version\":\"1.0\"}"
  Adapter1 : Subsystem
      settings: PortSchema="{\"entries\":[{\"content\":{\"margin\":10,\"minimumSpacing\":15,\"sides\":[{\"content\":{\"connectorIds\":[\"In1\",\"In2\",\"In3\",\"In4\"]},\"type\":\"ConnectorPlacement.EquallySpacedRectSide\",\"uuid\":\"0d9fb8ed-dc34-468d-b76e-34d51d64a929\"},{\"content\":{\"connectorIds\":[\"Out1\"],\"side\":\"RIGHT\"},\"type\":\"ConnectorPlacement.EquallySpacedRectSide\",\"uuid\":\"3640ebdc-29ef-4736-b1f3-b11a5268a051\"},{\"content\":{\"connectorIds\":[],\"side\":\"TOP\"},\"type\":\"ConnectorPlacement.EquallySpacedRectSide\",\"uuid\":\"ee7dc95f-9ee4-4519-b423-ed00e53cf3e5\"}]},\"type\":\"ConnectorPlacement.EquallySpacedConnector\",\"uuid\":\"5502122b-b863-467a-b80b-8b9d26248ea6\"}],\"packageUris\":[\"http://schema.mathworks.com/mf0/Connector/R2020b\"],\"version\":\"1.0\"}"
  Magnetotorquer 1 : Subsystem
      settings: PortSchema="{\"entries\":[{\"content\":{\"headerSize\":26,\"margin\":15,\"minimumSpacing\":25,\"sides\":[{\"content\":{\"connectorIds\":[\"In1\",\"In2\"]},\"type\":\"ConnectorPlacement.EquallySpacedRectSide\",\"uuid\":\"0d9fb8ed-dc34-468d-b76e-34d51d64a929\"},{\"content\":{\"connectorIds\":[\"Out1\",\"Out2\"],\"side\":\"RIGHT\"},\"type\":\"ConnectorPlacement.EquallySpacedRectSide\",\"uuid\":\"3640ebdc-29ef-4736-b1f3-b11a5268a051\"},{\"content\":{\"connectorIds\":[],\"side\":\"TOP\"},\"type\":\"ConnectorPlacement.EquallySpacedRectSide\",\"uuid\":\"ee7dc95f-9ee4-4519-b423-ed00e53cf3e5\"}]},\"type\":\"ConnectorPlacement.EquallySpacedConnector\",\"uuid\":\"5502122b-b863-467a-b80b-8b9d26248ea6\"}],\"packageUris\":[\"http://schema.mathworks.com/mf0/Connector/R2020b\"],\"version\":\"1.0\"}"
  Magnetotorquer 2 : Subsystem
      settings: PortSchema="{\"entries\":[{\"content\":{\"headerSize\":26,\"margin\":15,\"minimumSpacing\":25,\"sides\":[{\"content\":{\"connectorIds\":[\"In1\",\"In2\"]},\"type\":\"ConnectorPlacement.EquallySpacedRectSide\",\"uuid\":\"0d9fb8ed-dc34-468d-b76e-34d51d64a929\"},{\"content\":{\"connectorIds\":[\"Out1\",\"Out2\"],\"side\":\"RIGHT\"},\"type\":\"ConnectorPlacement.EquallySpacedRectSide\",\"uuid\":\"3640ebdc-29ef-4736-b1f3-b11a5268a051\"},{\"content\":{\"connectorIds\":[],\"side\":\"TOP\"},\"type\":\"ConnectorPlacement.EquallySpacedRectSide\",\"uuid\":\"ee7dc95f-9ee4-4519-b423-ed00e53cf3e5\"}]},\"type\":\"ConnectorPlacement.EquallySpacedConnector\",\"uuid\":\"5502122b-b863-467a-b80b-8b9d26248ea6\"}],\"packageUris\":[\"http://schema.mathworks.com/mf0/Connector/R2020b\"],\"version\":\"1.0\"}"
  Magnetotorquer 3 : Subsystem
      settings: PortSchema="{\"entries\":[{\"content\":{\"headerSize\":26,\"margin\":15,\"minimumSpacing\":25,\"sides\":[{\"content\":{\"connectorIds\":[\"In1\",\"In2\"]},\"type\":\"ConnectorPlacement.EquallySpacedRectSide\",\"uuid\":\"0d9fb8ed-dc34-468d-b76e-34d51d64a929\"},{\"content\":{\"connectorIds\":[\"Out1\",\"Out2\"],\"side\":\"RIGHT\"},\"type\":\"ConnectorPlacement.EquallySpacedRectSide\",\"uuid\":\"3640ebdc-29ef-4736-b1f3-b11a5268a051\"},{\"content\":{\"connectorIds\":[],\"side\":\"TOP\"},\"type\":\"ConnectorPlacement.EquallySpacedRectSide\",\"uuid\":\"ee7dc95f-9ee4-4519-b423-ed00e53cf3e5\"}]},\"type\":\"ConnectorPlacement.EquallySpacedConnector\",\"uuid\":\"5502122b-b863-467a-b80b-8b9d26248ea6\"}],\"packageUris\":[\"http://schema.mathworks.com/mf0/Connector/R2020b\"],\"version\":\"1.0\"}"
  Magnetotorquer 4 : Subsystem
      settings: PortSchema="{\"entries\":[{\"content\":{\"headerSize\":26,\"margin\":15,\"minimumSpacing\":25,\"sides\":[{\"content\":{\"connectorIds\":[\"In1\",\"In2\"]},\"type\":\"ConnectorPlacement.EquallySpacedRectSide\",\"uuid\":\"0d9fb8ed-dc34-468d-b76e-34d51d64a929\"},{\"content\":{\"connectorIds\":[\"Out1\",\"Out2\"],\"side\":\"RIGHT\"},\"type\":\"ConnectorPlacement.EquallySpacedRectSide\",\"uuid\":\"3640ebdc-29ef-4736-b1f3-b11a5268a051\"},{\"content\":{\"connectorIds\":[],\"side\":\"TOP\"},\"type\":\"ConnectorPlacement.EquallySpacedRectSide\",\"uuid\":\"ee7dc95f-9ee4-4519-b423-ed00e53cf3e5\"}]},\"type\":\"ConnectorPlacement.EquallySpacedConnector\",\"uuid\":\"5502122b-b863-467a-b80b-8b9d26248ea6\"}],\"packageUris\":[\"http://schema.mathworks.com/mf0/Connector/R2020b\"],\"version\":\"1.0\"}"
  Bus Element Out1 : Outport  PortName=Coil_Heat
  Bus Element Out2 : Outport  Port=2  PortName=Magnetic_Torque
  wires:
  Magnetotorquer 1/1(Heat 1) -> Adapter/1(Heat 1)
  Magnetotorquer 2/1(Heat 2) -> Adapter/2(Heat 2)
  Adapter/1(Coil_Heat) -> Bus Element Out1/1
  Magnetotorquer 3/1(Heat 3) -> Adapter/3(Heat 3)
  Magnetotorquer 4/1(Heat 4) -> Adapter/4(Heat 4)
  Magnetotorquer 1/2(Torque 1) -> Adapter1/1(Torque 1)
  Adapter1/1(Magnetic_Torque) -> Bus Element Out2/1
  Magnetotorquer 2/2(Torque 2) -> Adapter1/2(Torque 2)
  Magnetotorquer 3/2(Torque 3) -> Adapter1/3(Torque 3)
  Magnetotorquer 4/2(Torque 4) -> Adapter1/4(Torque 4)
  Bus Element In1/1 -> Magnetotorquer 1/1(Power)
  Bus Element In3/1 -> Magnetotorquer 2/1(Power)
  Bus Element In4/1 -> Magnetotorquer 3/1(Power)
  Bus Element In5/1 -> Magnetotorquer 4/1(Power)
  Bus Element In6/1 -> Magnetotorquer 2/2(Signal)
  Bus Element In7/1 -> Magnetotorquer 3/2(Signal)
  Bus Element In8/1 -> Magnetotorquer 4/2(Signal)
  Bus Element In2/1 -> Magnetotorquer 1/2(Signal)

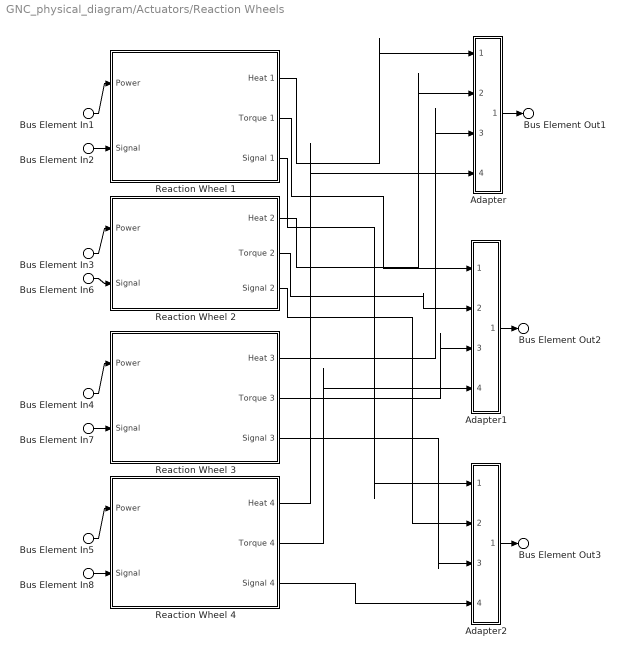
== system GNC_physical_diagram/Actuators/Reaction Wheels ==
  Bus Element In{1,3..5} (4 alike) : Inport  PortName=Power
  Bus Element In2 : Inport  Port=2  PortName=Signal  Element=Reaction_Wheel_1_Signal
  Bus Element In6 : Inport  Port=2  PortName=Signal  Element=Reaction_Wheel_2_Signa
  Bus Element In7 : Inport  Port=2  PortName=Signal  Element=Reaction_Wheel_3_Signa
  Bus Element In8 : Inport  Port=2  PortName=Signal  Element=Reaction_Wheel_4_Signa
  Adapter : Subsystem
      settings: PortSchema="{\"entries\":[{\"content\":{\"margin\":10,\"minimumSpacing\":15,\"sides\":[{\"content\":{\"connectorIds\":[\"In1\",\"In2\",\"In3\",\"In4\"]},\"type\":\"ConnectorPlacement.EquallySpacedRectSide\",\"uuid\":\"0d9fb8ed-dc34-468d-b76e-34d51d64a929\"},{\"content\":{\"connectorIds\":[\"Out1\"],\"side\":\"RIGHT\"},\"type\":\"ConnectorPlacement.EquallySpacedRectSide\",\"uuid\":\"3640ebdc-29ef-4736-b1f3-b11a5268a051\"},{\"content\":{\"connectorIds\":[],\"side\":\"TOP\"},\"type\":\"ConnectorPlacement.EquallySpacedRectSide\",\"uuid\":\"ee7dc95f-9ee4-4519-b423-ed00e53cf3e5\"}]},\"type\":\"ConnectorPlacement.EquallySpacedConnector\",\"uuid\":\"5502122b-b863-467a-b80b-8b9d26248ea6\"}],\"packageUris\":[\"http://schema.mathworks.com/mf0/Connector/R2020b\"],\"version\":\"1.0\"}"
  Adapter1 : Subsystem
      settings: PortSchema="{\"entries\":[{\"content\":{\"margin\":10,\"minimumSpacing\":15,\"sides\":[{\"content\":{\"connectorIds\":[\"In1\",\"In2\",\"In3\",\"In4\"]},\"type\":\"ConnectorPlacement.EquallySpacedRectSide\",\"uuid\":\"0d9fb8ed-dc34-468d-b76e-34d51d64a929\"},{\"content\":{\"connectorIds\":[\"Out1\"],\"side\":\"RIGHT\"},\"type\":\"ConnectorPlacement.EquallySpacedRectSide\",\"uuid\":\"3640ebdc-29ef-4736-b1f3-b11a5268a051\"},{\"content\":{\"connectorIds\":[],\"side\":\"TOP\"},\"type\":\"ConnectorPlacement.EquallySpacedRectSide\",\"uuid\":\"ee7dc95f-9ee4-4519-b423-ed00e53cf3e5\"}]},\"type\":\"ConnectorPlacement.EquallySpacedConnector\",\"uuid\":\"5502122b-b863-467a-b80b-8b9d26248ea6\"}],\"packageUris\":[\"http://schema.mathworks.com/mf0/Connector/R2020b\"],\"version\":\"1.0\"}"
  Adapter2 : Subsystem
      settings: PortSchema="{\"entries\":[{\"content\":{\"margin\":10,\"minimumSpacing\":15,\"sides\":[{\"content\":{\"connectorIds\":[\"In1\",\"In2\",\"In3\",\"In4\"]},\"type\":\"ConnectorPlacement.EquallySpacedRectSide\",\"uuid\":\"0d9fb8ed-dc34-468d-b76e-34d51d64a929\"},{\"content\":{\"connectorIds\":[\"Out1\"],\"side\":\"RIGHT\"},\"type\":\"ConnectorPlacement.EquallySpacedRectSide\",\"uuid\":\"3640ebdc-29ef-4736-b1f3-b11a5268a051\"},{\"content\":{\"connectorIds\":[],\"side\":\"TOP\"},\"type\":\"ConnectorPlacement.EquallySpacedRectSide\",\"uuid\":\"ee7dc95f-9ee4-4519-b423-ed00e53cf3e5\"}]},\"type\":\"ConnectorPlacement.EquallySpacedConnector\",\"uuid\":\"5502122b-b863-467a-b80b-8b9d26248ea6\"}],\"packageUris\":[\"http://schema.mathworks.com/mf0/Connector/R2020b\"],\"version\":\"1.0\"}"
  Reaction Wheel 1 : Subsystem
      settings: PortSchema="{\"entries\":[{\"content\":{\"headerSize\":26,\"margin\":15,\"minimumSpacing\":25,\"sides\":[{\"content\":{\"connectorIds\":[\"In1\",\"In2\"]},\"type\":\"ConnectorPlacement.EquallySpacedRectSide\",\"uuid\":\"0d9fb8ed-dc34-468d-b76e-34d51d64a929\"},{\"content\":{\"connectorIds\":[\"Out1\",\"Out2\",\"Out3\"],\"side\":\"RIGHT\"},\"type\":\"ConnectorPlacement.EquallySpacedRectSide\",\"uuid\":\"3640ebdc-29ef-4736-b1f3-b11a5268a051\"},{\"content\":{\"connectorIds\":[],\"side\":\"TOP\"},\"type\":\"ConnectorPlacement.EquallySpacedRectSide\",\"uuid\":\"ee7dc95f-9ee4-4519-b423-ed00e53cf3e5\"}]},\"type\":\"ConnectorPlacement.EquallySpacedConnector\",\"uuid\":\"5502122b-b863-467a-b80b-8b9d26248ea6\"}],\"packageUris\":[\"http://schema.mathworks.com/mf0/Connector/R2020b\"],\"version\":\"1.0\"}"
  Reaction Wheel 2 : Subsystem
      settings: PortSchema="{\"entries\":[{\"content\":{\"headerSize\":26,\"margin\":15,\"minimumSpacing\":25,\"sides\":[{\"content\":{\"connectorIds\":[\"In1\",\"In2\"]},\"type\":\"ConnectorPlacement.EquallySpacedRectSide\",\"uuid\":\"0d9fb8ed-dc34-468d-b76e-34d51d64a929\"},{\"content\":{\"connectorIds\":[\"Out1\",\"Out2\",\"Out3\"],\"side\":\"RIGHT\"},\"type\":\"ConnectorPlacement.EquallySpacedRectSide\",\"uuid\":\"3640ebdc-29ef-4736-b1f3-b11a5268a051\"},{\"content\":{\"connectorIds\":[],\"side\":\"TOP\"},\"type\":\"ConnectorPlacement.EquallySpacedRectSide\",\"uuid\":\"ee7dc95f-9ee4-4519-b423-ed00e53cf3e5\"}]},\"type\":\"ConnectorPlacement.EquallySpacedConnector\",\"uuid\":\"5502122b-b863-467a-b80b-8b9d26248ea6\"}],\"packageUris\":[\"http://schema.mathworks.com/mf0/Connector/R2020b\"],\"version\":\"1.0\"}"
  Reaction Wheel 3 : Subsystem
      settings: PortSchema="{\"entries\":[{\"content\":{\"headerSize\":26,\"margin\":15,\"minimumSpacing\":25,\"sides\":[{\"content\":{\"connectorIds\":[\"In1\",\"In2\"]},\"type\":\"ConnectorPlacement.EquallySpacedRectSide\",\"uuid\":\"0d9fb8ed-dc34-468d-b76e-34d51d64a929\"},{\"content\":{\"connectorIds\":[\"Out1\",\"Out2\",\"Out3\"],\"side\":\"RIGHT\"},\"type\":\"ConnectorPlacement.EquallySpacedRectSide\",\"uuid\":\"3640ebdc-29ef-4736-b1f3-b11a5268a051\"},{\"content\":{\"connectorIds\":[],\"side\":\"TOP\"},\"type\":\"ConnectorPlacement.EquallySpacedRectSide\",\"uuid\":\"ee7dc95f-9ee4-4519-b423-ed00e53cf3e5\"}]},\"type\":\"ConnectorPlacement.EquallySpacedConnector\",\"uuid\":\"5502122b-b863-467a-b80b-8b9d26248ea6\"}],\"packageUris\":[\"http://schema.mathworks.com/mf0/Connector/R2020b\"],\"version\":\"1.0\"}"
  Reaction Wheel 4 : Subsystem
      settings: PortSchema="{\"entries\":[{\"content\":{\"headerSize\":26,\"margin\":15,\"minimumSpacing\":25,\"sides\":[{\"content\":{\"connectorIds\":[\"In1\",\"In2\"]},\"type\":\"ConnectorPlacement.EquallySpacedRectSide\",\"uuid\":\"0d9fb8ed-dc34-468d-b76e-34d51d64a929\"},{\"content\":{\"connectorIds\":[\"Out1\",\"Out2\",\"Out3\"],\"side\":\"RIGHT\"},\"type\":\"ConnectorPlacement.EquallySpacedRectSide\",\"uuid\":\"3640ebdc-29ef-4736-b1f3-b11a5268a051\"},{\"content\":{\"connectorIds\":[],\"side\":\"TOP\"},\"type\":\"ConnectorPlacement.EquallySpacedRectSide\",\"uuid\":\"ee7dc95f-9ee4-4519-b423-ed00e53cf3e5\"}]},\"type\":\"ConnectorPlacement.EquallySpacedConnector\",\"uuid\":\"5502122b-b863-467a-b80b-8b9d26248ea6\"}],\"packageUris\":[\"http://schema.mathworks.com/mf0/Connector/R2020b\"],\"version\":\"1.0\"}"
  Bus Element Out1 : Outport  PortName=Motor_Heat
  Bus Element Out2 : Outport  Port=2  PortName=Reaction_Torque
  Bus Element Out3 : Outport  Port=3  PortName=Encoder Signal
  wires:
  Adapter/1(Motor_Heat) -> Bus Element Out1/1
  Reaction Wheel 1/1(Heat 1) -> Adapter/1(Heat 1)
  Reaction Wheel 2/1(Heat 2) -> Adapter/2(Heat 2)
  Reaction Wheel 3/1(Heat 3) -> Adapter/3(Heat 3)
  Reaction Wheel 4/1(Heat 4) -> Adapter/4(Heat 4)
  Adapter1/1(Reaction_Torque) -> Bus Element Out2/1
  Reaction Wheel 1/2(Torque 1) -> Adapter1/1(Torque 1)
  Reaction Wheel 2/2(Torque 2) -> Adapter1/2(Torque 2)
  Reaction Wheel 3/2(Torque 3) -> Adapter1/3(Torque 4)
  Reaction Wheel 4/2(Torque 4) -> Adapter1/4(InBus)
  Adapter2/1(Encoder Signal) -> Bus Element Out3/1
  Reaction Wheel 1/3(Signal 1) -> Adapter2/1(Signal 1)
  Reaction Wheel 2/3(Signal 2) -> Adapter2/2(Signal 2)
  Reaction Wheel 3/3(Signal 3) -> Adapter2/3(Signal 3)
  Reaction Wheel 4/3(Signal 4) -> Adapter2/4(Signal 4)
  Bus Element In1/1 -> Reaction Wheel 1/1(Power)
  Bus Element In3/1 -> Reaction Wheel 2/1(Power)
  Bus Element In4/1 -> Reaction Wheel 3/1(Power)
  Bus Element In5/1 -> Reaction Wheel 4/1(Power)
  Bus Element In2/1 -> Reaction Wheel 1/2(Signal)
  Bus Element In6/1 -> Reaction Wheel 2/2(Signal)
  Bus Element In7/1 -> Reaction Wheel 3/2(Signal)
  Bus Element In8/1 -> Reaction Wheel 4/2(Signal)

== system GNC_physical_diagram/Avionics Hardware/Ground Station ==
  Bus Element In1 : Inport  PortName=Controller Data
  Bus Element In2 : Inport  Port=2  PortName=Orientation Estimation
  Bus Element In3 : Inport  Port=3  PortName=Data Stream
  Trajectory Estimation : Subsystem
      settings: PortSchema="{\"entries\":[{\"content\":{\"headerSize\":26,\"margin\":15,\"minimumSpacing\":25,\"sides\":[{\"content\":{\"connectorIds\":[\"In1\",\"In2\"]},\"type\":\"ConnectorPlacement.EquallySpacedRectSide\",\"uuid\":\"84b5d53f-2022-465e-8fea-a5f6f770027c\"},{\"content\":{\"connectorIds\":[\"Out1\"],\"side\":\"RIGHT\"},\"type\":\"ConnectorPlacement.EquallySpacedRectSide\",\"uuid\":\"3040b22b-4da9-4e90-8b1d-cb2b07104062\"},{\"content\":{\"connectorIds\":[],\"side\":\"TOP\"},\"type\":\"ConnectorPlacement.EquallySpacedRectSide\",\"uuid\":\"0c703596-6fc3-4e59-bd9e-7a374b07bd61\"}]},\"type\":\"ConnectorPlacement.EquallySpacedConnector\",\"uuid\":\"5254ac91-cce0-48ff-acfe-a25b2e5a66da\"}],\"packageUris\":[\"http://schema.mathworks.com/mf0/Connector/R2020b\"],\"version\":\"1.0\"}"
  Bus Element Out1 : Outport  PortName=Tunable Gains
  wires:
  Bus Element In3/1 -> Trajectory Estimation/2(Loggable Data)
  Bus Element In2/1 -> Trajectory Estimation/1(Orientation Estimation)

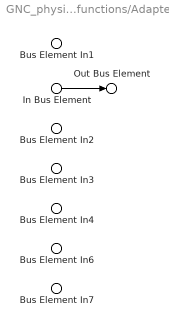
== system GNC_physical_diagram/GNC functions/Adapter ==
  In Bus Element : Inport  PortName=Detumbling_Done
  Bus Element In1 : Inport  Port=2  PortName=Maintaining
  Bus Element In2 : Inport  Port=3  PortName=Rotation_Done
  Bus Element In3 : Inport  Port=4  PortName=Is_Rotating
  Bus Element In4 : Inport  Port=5  PortName=Testing_Done
  Bus Element In6 : Inport  Port=6  PortName=Recreation_Done
  Bus Element In7 : Inport  Port=7  PortName=GNC_Turned_off
  Out Bus Element : Outport  PortName=GNC_Status_
  wires:
  In Bus Element/1 -> Out Bus Element/1

== system GNC_physical_diagram/GNC functions/Deorbiting ==
  Bus Element In1 : Inport  PortName=Trigger
  Bus Element Out1 : Outport  PortName=GNC_Turned_off

== system GNC_physical_diagram/GNC functions/Detumbling ==
  Bus Element In1 : Inport  PortName=Orientation Estimation
  Bus Element In5 : Inport  Port=2  PortName=Trigger
  Bus Element In6 : Inport  Port=3  PortName=Requires_Actuators
  Bus Element In4 : Inport  Port=4  PortName=Resource_Budget
  Bus Element Out1 : Outport  PortName=Detumbling_Done
